simulink model "dx_hand_model"  (R2017b)
settings: Solver=ode3  StartTime=0.0  StopTime=inf  FixedStep=0.01  RelTol=1e-3  EnableMultiTasking=on
InitFcn:
  | cutFreq = 0.1; % T
  | sampleTime = 0.01;
  | filt = tf(1,[cutFreq 1]);
  | filt = c2d(filt,sampleTime);
  | 
  | cutFreq2 = 1;
  | filt2 = tf(1,[cutFreq2 1]);
  | filt2 = c2d(filt2,sampleTime);
  | 
  | cutFreq3 = 0.3;
  | filt3 = tf(1,[cutFreq3 1]);
  | filt3 = c2d(filt3,sampleTime);
  | 
  | update_param = 2;
  | 
  | ampliFactor = 1.60;
  | ampliFactorMiddle = 2.00;
  | ampliFactorDistal = 1;
  | 
  | % Set Hand Address
  | % RightHandAddress = '10.100.39.144';
  | RightHandAddress = '10.24.4.91';
  | Verosim = '10.100.39.22'
  | LeftHandAddress = '10.100.39.22'
  | 
  | max_force = 24; % Newton
model workspace (MAT data in the model file):
  SL_ROS_VariableLengthArrays_MaxSizes : struct (value not decoded)
libraries: robotlib x136, simulink_extras x27, simulink x16, etargetslib x2, dspnetwork x2
(part 16 of 19)

== matlab function dx_hand_model/Thumb/Proximal and Distal Phalanx/Find K ==
  data: PIP input; x_sol output; G2 input; G1 input; s2 input; y_sol output; z_sol output
function [x_sol,y_sol,z_sol] = sysEqn(PIP, G2, G1,s2)
CMC = PIP;
F = G2;
F_1 = G1;
s1 = s2;
CMC1 = CMC(1);
CMC2 = CMC(2);
CMC3 = CMC(3);
F1 = F(1);
F2 =F(2);
F3 = F(3);
F_11 = F_1(1);
F_12 = F_1(2);
F_13 = F_1(3);
%SYSEQNOPTIMIZED
%    [X_SOL,Y_SOL,Z_SOL] = SYSEQNOPTIMIZED(CMC1,CMC2,CMC3,F1,F2,F3,F_11,F_12,F_13,S1)

%    This function was generated by the Symbolic Math Toolbox version 8.0.
%    24-Jan-2018 17:02:07

t2 = CMC1.^2;
t3 = CMC2.^2;
t4 = F1.^2;
t5 = F2.^2;
t6 = F3.^2;
t7 = CMC3.^2;
t8 = s1.^2;
t21 = CMC1.*F1.*2.0;
t22 = CMC2.*F2.*2.0;
t23 = CMC3.*F3.*2.0;
t9 = t2+t3+t4+t5+t6+t7-t21-t22-t23;
t25 = F3.*t2;
t26 = F3.*t3;
t27 = CMC3.*t6.*2.0;
t28 = F3.*t7;
t29 = F3.*t4;
t30 = F3.*t5;
t31 = CMC3.*t8;
t32 = F3.*t8;
t33 = CMC1.*F1.*F3.*2.0;
t34 = CMC2.*F2.*F3.*2.0;
t1256 = F3.*t6;
t10 = t25+t26-t27+t28+t29+t30+t31-t32-t33-t34+t1256;
t11 = t2.^2;
t12 = t4.^2;
t13 = t6.^2;
t14 = t5.^2;
t15 = t3.^2;
t16 = t7.^2;
t17 = F_11.^2;
t18 = F_13.^2;
t19 = F_12.^2;
t20 = t8.^2;
t24 = 1.0./t9.^2;
t35 = t10.^2;
t36 = t24.*t35;
t37 = t2.*t14;
t38 = t3.*t12;
t39 = t5.*t11;
t40 = t4.*t15;
t41 = t2.*t13;
t42 = t6.*t11;
t43 = t7.*t12;
t44 = t4.*t16;
t45 = t3.*t13;
t46 = t7.*t14;
t47 = t6.*t15;
t48 = t5.*t16;
t49 = t11.*t19;
t50 = t15.*t17;
t51 = t11.*t18;
t52 = t16.*t17;
t53 = t15.*t18;
t54 = t16.*t19;
t55 = t12.*t19;
t56 = t14.*t17;
t57 = t12.*t18;
t58 = t13.*t17;
t59 = t14.*t18;
t60 = t13.*t19;
t61 = t2.*t3.*t4;
t62 = t2.*t3.*t5;
t63 = t2.*t4.*t7;
t64 = t2.*t3.*t6.*2.0;
t65 = t2.*t5.*t7.*2.0;
t66 = t3.*t4.*t7.*2.0;
t67 = t2.*t6.*t7;
t68 = t3.*t5.*t7;
t69 = t3.*t6.*t7;
t70 = t2.*t3.*t17;
t71 = t2.*t3.*t19;
t72 = t2.*t7.*t17;
t73 = t2.*t3.*t18.*2.0;
t74 = t2.*t7.*t19.*2.0;
t75 = t3.*t7.*t17.*2.0;
t76 = t2.*t7.*t18;
t77 = t3.*t7.*t19;
t78 = t3.*t7.*t18;
t79 = t2.*t4.*t5;
t80 = t2.*t4.*t6;
t81 = t3.*t4.*t5;
t82 = t2.*t5.*t6.*2.0;
t83 = t3.*t4.*t6.*2.0;
t84 = t4.*t5.*t7.*2.0;
t85 = t3.*t5.*t6;
t86 = t4.*t6.*t7;
t87 = t5.*t6.*t7;
t88 = t2.*t4.*t19.*6.0;
t89 = t2.*t5.*t17;
t90 = t3.*t4.*t17;
t91 = t2.*t4.*t18.*6.0;
t92 = t2.*t5.*t19;
t93 = t2.*t6.*t17;
t94 = t3.*t4.*t19;
t95 = t3.*t5.*t17.*6.0;
t96 = t4.*t7.*t17;
t97 = t2.*t5.*t18.*2.0;
t98 = t2.*t6.*t19.*2.0;
t99 = t3.*t4.*t18.*2.0;
t100 = t3.*t6.*t17.*2.0;
t101 = t4.*t7.*t19.*2.0;
t102 = t5.*t7.*t17.*2.0;
t103 = t2.*t6.*t18;
t104 = t3.*t5.*t18.*6.0;
t105 = t3.*t6.*t19;
t106 = t4.*t7.*t18;
t107 = t5.*t7.*t19;
t108 = t6.*t7.*t17.*6.0;
t109 = t3.*t6.*t18;
t110 = t5.*t7.*t18;
t111 = t6.*t7.*t19.*6.0;
t112 = t4.*t5.*t17;
t113 = t4.*t5.*t19;
t114 = t4.*t6.*t17;
t115 = t4.*t5.*t18.*2.0;
t116 = t4.*t6.*t19.*2.0;
t117 = t5.*t6.*t17.*2.0;
t118 = t4.*t6.*t18;
t119 = t5.*t6.*t19;
t120 = t5.*t6.*t18;
t121 = CMC1.*F1.*t3.*t5.*4.0;
t122 = CMC2.*F2.*t2.*t4.*4.0;
t123 = CMC1.*F1.*t6.*t7.*4.0;
t124 = CMC3.*F3.*t2.*t4.*4.0;
t125 = CMC2.*F2.*t6.*t7.*4.0;
t126 = CMC3.*F3.*t3.*t5.*4.0;
t127 = CMC1.*F_11.*t3.*t4.*4.0;
t128 = CMC1.*F_11.*t4.*t7.*4.0;
t129 = CMC2.*F_12.*t2.*t5.*4.0;
t130 = CMC2.*F_12.*t5.*t7.*4.0;
t131 = CMC3.*F_13.*t2.*t6.*4.0;
t132 = CMC3.*F_13.*t3.*t6.*4.0;
t133 = F1.*F_11.*t2.*t5.*4.0;
t134 = F1.*F_11.*t2.*t6.*4.0;
t135 = F2.*F_12.*t3.*t4.*4.0;
t136 = F2.*F_12.*t3.*t6.*4.0;
t137 = F3.*F_13.*t4.*t7.*4.0;
t138 = F3.*F_13.*t5.*t7.*4.0;
t139 = CMC1.*CMC2.*F1.*F_12.*t4.*6.0;
t140 = CMC1.*CMC2.*F2.*F_11.*t5.*6.0;
t141 = CMC1.*CMC2.*F1.*F_12.*t3.*2.0;
t142 = CMC1.*CMC2.*F2.*F_11.*t3.*2.0;
t143 = CMC1.*CMC2.*F1.*F_12.*t2.*2.0;
t144 = CMC1.*CMC2.*F2.*F_11.*t2.*2.0;
t145 = CMC1.*CMC3.*F1.*F_13.*t4.*6.0;
t146 = CMC1.*CMC3.*F3.*F_11.*t6.*6.0;
t147 = CMC1.*CMC3.*F1.*F_13.*t7.*2.0;
t148 = CMC1.*CMC3.*F3.*F_11.*t7.*2.0;
t149 = CMC1.*CMC3.*F1.*F_13.*t2.*2.0;
t150 = CMC1.*CMC3.*F3.*F_11.*t2.*2.0;
t151 = CMC2.*CMC3.*F2.*F_13.*t5.*6.0;
t152 = CMC2.*CMC3.*F3.*F_12.*t6.*6.0;
t153 = CMC2.*CMC3.*F2.*F_13.*t7.*2.0;
t154 = CMC2.*CMC3.*F3.*F_12.*t7.*2.0;
t155 = CMC2.*CMC3.*F2.*F_13.*t3.*2.0;
t156 = CMC2.*CMC3.*F3.*F_12.*t3.*2.0;
t157 = CMC1.*F1.*F2.*F_12.*t5.*2.0;
t158 = CMC1.*F1.*F2.*F_12.*t4.*2.0;
t159 = CMC2.*F1.*F2.*F_11.*t5.*2.0;
t160 = CMC2.*F1.*F2.*F_11.*t4.*2.0;
t161 = CMC1.*F1.*F2.*F_12.*t2.*6.0;
t162 = CMC2.*F1.*F2.*F_11.*t3.*6.0;
t163 = CMC1.*F1.*F3.*F_13.*t6.*2.0;
t164 = CMC1.*F1.*F3.*F_13.*t4.*2.0;
t165 = CMC3.*F1.*F3.*F_11.*t6.*2.0;
t166 = CMC3.*F1.*F3.*F_11.*t4.*2.0;
t167 = CMC1.*F1.*F3.*F_13.*t2.*6.0;
t168 = CMC3.*F1.*F3.*F_11.*t7.*6.0;
t169 = CMC2.*F2.*F3.*F_13.*t6.*2.0;
t170 = CMC2.*F2.*F3.*F_13.*t5.*2.0;
t171 = CMC3.*F2.*F3.*F_12.*t6.*2.0;
t172 = CMC3.*F2.*F3.*F_12.*t5.*2.0;
t173 = CMC2.*F2.*F3.*F_13.*t3.*6.0;
t174 = CMC3.*F2.*F3.*F_12.*t7.*6.0;
t175 = CMC1.*F2.*F_11.*F_12.*t5.*2.0;
t176 = CMC2.*F1.*F_11.*F_12.*t4.*2.0;
t177 = CMC1.*F2.*F_11.*F_12.*t2.*2.0;
t178 = CMC2.*F1.*F_11.*F_12.*t3.*2.0;
t179 = CMC1.*F3.*F_11.*F_13.*t6.*2.0;
t180 = CMC3.*F1.*F_11.*F_13.*t4.*2.0;
t181 = CMC1.*F3.*F_11.*F_13.*t2.*2.0;
t182 = CMC3.*F1.*F_11.*F_13.*t7.*2.0;
t183 = CMC2.*F3.*F_12.*F_13.*t6.*2.0;
t184 = CMC3.*F2.*F_12.*F_13.*t5.*2.0;
t185 = CMC2.*F3.*F_12.*F_13.*t3.*2.0;
t186 = CMC3.*F2.*F_12.*F_13.*t7.*2.0;
t187 = CMC1.*CMC2.*F1.*F_12.*t7.*2.0;
t188 = CMC1.*CMC2.*F2.*F_11.*t7.*2.0;
t189 = CMC1.*CMC3.*F1.*F_13.*t3.*2.0;
t190 = CMC1.*CMC3.*F3.*F_11.*t3.*2.0;
t191 = CMC2.*CMC3.*F2.*F_13.*t2.*2.0;
t192 = CMC2.*CMC3.*F3.*F_12.*t2.*2.0;
t193 = CMC1.*CMC2.*F1.*F2.*t17.*4.0;
t194 = CMC1.*CMC2.*F1.*F2.*t19.*4.0;
t195 = CMC1.*CMC2.*F1.*F2.*t18.*8.0;
t196 = CMC1.*CMC2.*F1.*F_12.*t6.*6.0;
t197 = CMC1.*CMC2.*F2.*F_11.*t6.*6.0;
t198 = CMC1.*CMC3.*F1.*F3.*t17.*4.0;
t199 = CMC1.*F1.*F2.*F_12.*t7.*6.0;
t200 = CMC2.*F1.*F2.*F_11.*t7.*6.0;
t201 = CMC1.*CMC3.*F1.*F3.*t19.*8.0;
t202 = CMC1.*CMC3.*F1.*F_13.*t5.*6.0;
t203 = CMC1.*CMC3.*F3.*F_11.*t5.*6.0;
t204 = CMC1.*F1.*F3.*F_13.*t3.*6.0;
t205 = CMC3.*F1.*F3.*F_11.*t3.*6.0;
t206 = CMC1.*CMC3.*F1.*F3.*t18.*4.0;
t207 = CMC2.*CMC3.*F2.*F3.*t17.*8.0;
t208 = CMC2.*CMC3.*F2.*F_13.*t4.*6.0;
t209 = CMC2.*CMC3.*F3.*F_12.*t4.*6.0;
t210 = CMC2.*F2.*F3.*F_13.*t2.*6.0;
t211 = CMC3.*F2.*F3.*F_12.*t2.*6.0;
t212 = CMC2.*CMC3.*F2.*F3.*t19.*4.0;
t213 = CMC2.*CMC3.*F2.*F3.*t18.*4.0;
t214 = CMC2.*F1.*F_11.*F_12.*t2.*6.0;
t215 = CMC1.*F2.*F_11.*F_12.*t3.*6.0;
t216 = CMC1.*F2.*F_11.*F_12.*t7.*2.0;
t217 = CMC2.*F1.*F_11.*F_12.*t7.*2.0;
t218 = CMC3.*F1.*F_11.*F_13.*t2.*6.0;
t219 = CMC1.*F3.*F_11.*F_13.*t3.*2.0;
t220 = CMC3.*F1.*F_11.*F_13.*t3.*2.0;
t221 = CMC1.*F3.*F_11.*F_13.*t7.*6.0;
t222 = CMC2.*F3.*F_12.*F_13.*t2.*2.0;
t223 = CMC3.*F2.*F_12.*F_13.*t2.*2.0;
t224 = CMC3.*F2.*F_12.*F_13.*t3.*6.0;
t225 = CMC2.*F3.*F_12.*F_13.*t7.*6.0;
t226 = CMC1.*F1.*F2.*F_12.*t6.*2.0;
t227 = CMC2.*F1.*F2.*F_11.*t6.*2.0;
t228 = CMC1.*F1.*F3.*F_13.*t5.*2.0;
t229 = CMC3.*F1.*F3.*F_11.*t5.*2.0;
t230 = CMC2.*F2.*F3.*F_13.*t4.*2.0;
t231 = CMC3.*F2.*F3.*F_12.*t4.*2.0;
t232 = CMC1.*F2.*F_11.*F_12.*t4.*6.0;
t233 = CMC2.*F1.*F_11.*F_12.*t5.*6.0;
t234 = CMC1.*F2.*F_11.*F_12.*t6.*2.0;
t235 = CMC1.*F3.*F_11.*F_13.*t4.*6.0;
t236 = CMC2.*F1.*F_11.*F_12.*t6.*2.0;
t237 = CMC1.*F3.*F_11.*F_13.*t5.*2.0;
t238 = CMC3.*F1.*F_11.*F_13.*t5.*2.0;
t239 = CMC2.*F3.*F_12.*F_13.*t4.*2.0;
t240 = CMC3.*F1.*F_11.*F_13.*t6.*6.0;
t241 = CMC3.*F2.*F_12.*F_13.*t4.*2.0;
t242 = CMC2.*F3.*F_12.*F_13.*t5.*6.0;
t243 = CMC3.*F2.*F_12.*F_13.*t6.*6.0;
t244 = CMC1.*F1.*F2.*F3.*F_12.*F_13.*4.0;
t245 = CMC2.*F1.*F2.*F3.*F_11.*F_13.*4.0;
t246 = CMC3.*F1.*F2.*F3.*F_11.*F_12.*4.0;
t247 = CMC1.*CMC2.*CMC3.*F1.*F2.*F3.*1.2e1;
t248 = CMC1.*CMC2.*CMC3.*F1.*F_12.*F_13.*4.0;
t249 = CMC1.*CMC2.*CMC3.*F2.*F_11.*F_13.*4.0;
t250 = CMC1.*CMC2.*CMC3.*F3.*F_11.*F_12.*4.0;
t633 = CMC1.*F_11.*t14.*2.0;
t634 = F1.*F_11.*t15.*2.0;
t635 = CMC1.*F_11.*t13.*2.0;
t636 = CMC2.*F_12.*t12.*2.0;
t637 = F2.*F_12.*t11.*2.0;
t638 = F1.*F_11.*t16.*2.0;
t639 = CMC2.*F_12.*t13.*2.0;
t640 = CMC3.*F_13.*t12.*2.0;
t641 = F3.*F_13.*t11.*2.0;
t642 = F2.*F_12.*t16.*2.0;
t643 = CMC3.*F_13.*t14.*2.0;
t644 = F3.*F_13.*t15.*2.0;
t645 = CMC1.*F1.*t3.*t4.*2.0;
t646 = CMC1.*F1.*t4.*t7.*2.0;
t647 = CMC2.*F2.*t2.*t5.*2.0;
t648 = CMC2.*F2.*t5.*t7.*2.0;
t649 = CMC3.*F3.*t2.*t6.*2.0;
t650 = CMC3.*F3.*t3.*t6.*2.0;
t651 = CMC1.*F1.*t2.*t5.*2.0;
t652 = CMC1.*F1.*t2.*t6.*2.0;
t653 = CMC2.*F2.*t3.*t4.*2.0;
t654 = CMC2.*F2.*t3.*t6.*2.0;
t655 = CMC3.*F3.*t4.*t7.*2.0;
t656 = CMC3.*F3.*t5.*t7.*2.0;
t657 = CMC1.*F1.*t4.*t19.*4.0;
t658 = CMC1.*F1.*t2.*t19.*4.0;
t659 = CMC1.*F_11.*t2.*t5.*2.0;
t660 = F1.*F_11.*t3.*t4.*2.0;
t661 = CMC1.*F1.*t4.*t18.*4.0;
t662 = CMC2.*F2.*t5.*t17.*4.0;
t663 = F2.*F_12.*t2.*t5.*2.0;
t664 = CMC1.*F1.*t2.*t18.*4.0;
t665 = CMC1.*F_11.*t2.*t6.*2.0;
t666 = CMC2.*F2.*t3.*t17.*4.0;
t667 = CMC2.*F_12.*t3.*t4.*2.0;
t668 = F1.*F_11.*t4.*t7.*2.0;
t669 = CMC2.*F2.*t5.*t18.*4.0;
t670 = CMC3.*F3.*t6.*t17.*4.0;
t671 = F3.*F_13.*t2.*t6.*2.0;
t672 = CMC2.*F2.*t3.*t18.*4.0;
t673 = CMC2.*F_12.*t3.*t6.*2.0;
t674 = F2.*F_12.*t5.*t7.*2.0;
t675 = CMC3.*F3.*t7.*t17.*4.0;
t676 = CMC3.*F_13.*t4.*t7.*2.0;
t677 = CMC3.*F3.*t6.*t19.*4.0;
t678 = F3.*F_13.*t3.*t6.*2.0;
t679 = CMC3.*F3.*t7.*t19.*4.0;
t680 = CMC3.*F_13.*t5.*t7.*2.0;
t681 = CMC1.*F1.*t3.*t6.*2.0;
t682 = CMC1.*F1.*t5.*t7.*2.0;
t683 = CMC2.*F2.*t4.*t7.*2.0;
t684 = CMC2.*F2.*t2.*t6.*2.0;
t685 = CMC3.*F3.*t2.*t5.*2.0;
t686 = CMC3.*F3.*t3.*t4.*2.0;
t687 = CMC1.*F1.*t3.*t17.*2.0;
t688 = F1.*F_11.*t2.*t3.*2.0;
t689 = CMC1.*F1.*t3.*t19.*2.0;
t690 = CMC1.*F_11.*t3.*t5.*6.0;
t691 = CMC1.*F1.*t7.*t17.*2.0;
t692 = CMC2.*F2.*t2.*t17.*2.0;
t693 = CMC2.*F_12.*t2.*t4.*6.0;
t694 = F1.*F_11.*t2.*t7.*2.0;
t695 = CMC1.*F1.*t3.*t18.*4.0;
t696 = CMC1.*F_11.*t3.*t6.*2.0;
t697 = CMC1.*F1.*t7.*t19.*4.0;
t698 = CMC1.*F_11.*t5.*t7.*2.0;
t699 = CMC2.*F2.*t2.*t19.*2.0;
t700 = F2.*F_12.*t2.*t3.*2.0;
t701 = F1.*F_11.*t3.*t7.*4.0;
t702 = CMC1.*F1.*t7.*t18.*2.0;
t703 = CMC1.*F_11.*t6.*t7.*6.0;
t704 = CMC2.*F2.*t7.*t17.*4.0;
t705 = CMC2.*F_12.*t4.*t7.*2.0;
t706 = CMC2.*F2.*t2.*t18.*4.0;
t707 = CMC2.*F_12.*t2.*t6.*2.0;
t708 = CMC3.*F3.*t2.*t17.*2.0;
t709 = CMC3.*F_13.*t2.*t4.*6.0;
t710 = F2.*F_12.*t2.*t7.*4.0;
t711 = CMC2.*F2.*t7.*t19.*2.0;
t712 = CMC3.*F3.*t2.*t19.*4.0;
t713 = CMC3.*F_13.*t2.*t5.*2.0;
t714 = F3.*F_13.*t2.*t3.*4.0;
t715 = CMC3.*F3.*t3.*t17.*4.0;
t716 = CMC3.*F_13.*t3.*t4.*2.0;
t717 = F2.*F_12.*t3.*t7.*2.0;
t718 = CMC2.*F2.*t7.*t18.*2.0;
t719 = CMC2.*F_12.*t6.*t7.*6.0;
t720 = CMC3.*F3.*t2.*t18.*2.0;
t721 = F3.*F_13.*t2.*t7.*2.0;
t722 = CMC3.*F3.*t3.*t19.*2.0;
t723 = CMC3.*F_13.*t3.*t5.*6.0;
t724 = CMC3.*F3.*t3.*t18.*2.0;
t725 = F3.*F_13.*t3.*t7.*2.0;
t726 = CMC1.*F1.*t5.*t17.*2.0;
t727 = CMC1.*F_11.*t4.*t5.*2.0;
t728 = CMC1.*F1.*t5.*t19.*2.0;
t729 = CMC1.*F1.*t6.*t17.*2.0;
t730 = CMC1.*F_11.*t4.*t6.*2.0;
t731 = CMC2.*F2.*t4.*t17.*2.0;
t732 = F2.*F_12.*t2.*t4.*6.0;
t733 = F1.*F_11.*t3.*t5.*6.0;
t734 = CMC1.*F1.*t5.*t18.*4.0;
t735 = CMC1.*F1.*t6.*t19.*4.0;
t736 = CMC1.*F_11.*t5.*t6.*4.0;
t737 = CMC2.*F2.*t4.*t19.*2.0;
t738 = CMC2.*F_12.*t4.*t5.*2.0;
t739 = F1.*F_11.*t3.*t6.*2.0;
t740 = F1.*F_11.*t5.*t7.*2.0;
t741 = CMC1.*F1.*t6.*t18.*2.0;
t742 = CMC2.*F2.*t6.*t17.*4.0;
t743 = CMC2.*F2.*t4.*t18.*4.0;
t744 = CMC2.*F_12.*t4.*t6.*4.0;
t745 = CMC3.*F3.*t4.*t17.*2.0;
t746 = F2.*F_12.*t2.*t6.*2.0;
t747 = F3.*F_13.*t2.*t4.*6.0;
t748 = F1.*F_11.*t6.*t7.*6.0;
t749 = F2.*F_12.*t4.*t7.*2.0;
t750 = CMC2.*F2.*t6.*t19.*2.0;
t751 = CMC2.*F_12.*t5.*t6.*2.0;
t752 = CMC3.*F3.*t4.*t19.*4.0;
t753 = CMC3.*F_13.*t4.*t5.*4.0;
t754 = CMC3.*F3.*t5.*t17.*4.0;
t755 = F3.*F_13.*t2.*t5.*2.0;
t756 = F3.*F_13.*t3.*t4.*2.0;
t757 = CMC2.*F2.*t6.*t18.*2.0;
t758 = CMC3.*F3.*t4.*t18.*2.0;
t759 = CMC3.*F_13.*t4.*t6.*2.0;
t760 = CMC3.*F3.*t5.*t19.*2.0;
t761 = F3.*F_13.*t3.*t5.*6.0;
t762 = F2.*F_12.*t6.*t7.*6.0;
t763 = CMC3.*F3.*t5.*t18.*2.0;
t764 = CMC3.*F_13.*t5.*t6.*2.0;
t765 = CMC1.*CMC2.*F1.*F2.*t5.*2.0;
t766 = CMC1.*CMC2.*F1.*F2.*t4.*2.0;
t767 = CMC1.*CMC2.*F1.*F2.*t3.*2.0;
t768 = CMC1.*CMC2.*F1.*F2.*t2.*2.0;
t769 = CMC1.*CMC3.*F1.*F3.*t6.*2.0;
t770 = CMC1.*CMC3.*F1.*F3.*t4.*2.0;
t771 = CMC1.*CMC3.*F1.*F3.*t7.*2.0;
t772 = CMC1.*CMC3.*F1.*F3.*t2.*2.0;
t773 = CMC2.*CMC3.*F2.*F3.*t6.*2.0;
t774 = CMC2.*CMC3.*F2.*F3.*t5.*2.0;
t775 = CMC2.*CMC3.*F2.*F3.*t7.*2.0;
t776 = CMC2.*CMC3.*F2.*F3.*t3.*2.0;
t777 = CMC1.*CMC2.*F_11.*F_12.*t3.*2.0;
t778 = CMC1.*CMC2.*F_11.*F_12.*t2.*2.0;
t779 = CMC1.*CMC3.*F_11.*F_13.*t7.*2.0;
t780 = CMC1.*CMC3.*F_11.*F_13.*t2.*2.0;
t781 = CMC2.*CMC3.*F_12.*F_13.*t7.*2.0;
t782 = CMC2.*CMC3.*F_12.*F_13.*t3.*2.0;
t783 = F1.*F2.*F_11.*F_12.*t5.*2.0;
t784 = F1.*F2.*F_11.*F_12.*t4.*2.0;
t785 = F1.*F3.*F_11.*F_13.*t6.*2.0;
t786 = F1.*F3.*F_11.*F_13.*t4.*2.0;
t787 = F2.*F3.*F_12.*F_13.*t6.*2.0;
t788 = F2.*F3.*F_12.*F_13.*t5.*2.0;
t789 = CMC1.*CMC2.*F1.*F2.*t7.*2.0;
t790 = CMC1.*CMC3.*F1.*F3.*t3.*2.0;
t791 = CMC2.*CMC3.*F2.*F3.*t2.*2.0;
t792 = CMC1.*CMC2.*F_11.*F_12.*t7.*2.0;
t793 = CMC1.*CMC3.*F_11.*F_13.*t3.*2.0;
t794 = CMC2.*CMC3.*F_12.*F_13.*t2.*2.0;
t795 = CMC1.*CMC2.*F1.*F2.*t6.*2.0;
t796 = CMC1.*CMC3.*F1.*F3.*t5.*2.0;
t797 = CMC2.*CMC3.*F2.*F3.*t4.*2.0;
t798 = CMC1.*CMC2.*F2.*F_11.*t4.*2.0;
t799 = CMC2.*F1.*F2.*F_11.*t2.*2.0;
t800 = CMC1.*CMC2.*F1.*F_12.*t5.*2.0;
t801 = CMC1.*F1.*F2.*F_12.*t3.*2.0;
t802 = CMC1.*CMC3.*F3.*F_11.*t4.*2.0;
t803 = CMC3.*F1.*F3.*F_11.*t2.*2.0;
t804 = CMC1.*CMC3.*F1.*F_13.*t6.*2.0;
t805 = CMC1.*F1.*F3.*F_13.*t7.*2.0;
t806 = CMC2.*CMC3.*F3.*F_12.*t5.*2.0;
t807 = CMC3.*F2.*F3.*F_12.*t3.*2.0;
t808 = CMC2.*CMC3.*F2.*F_13.*t6.*2.0;
t809 = CMC2.*F2.*F3.*F_13.*t7.*2.0;
t810 = CMC1.*CMC2.*F_11.*F_12.*t4.*6.0;
t811 = CMC1.*CMC2.*F_11.*F_12.*t5.*6.0;
t812 = CMC1.*CMC2.*F_11.*F_12.*t6.*2.0;
t813 = CMC1.*CMC3.*F_11.*F_13.*t4.*6.0;
t814 = CMC1.*CMC3.*F_11.*F_13.*t5.*2.0;
t815 = CMC1.*CMC3.*F_11.*F_13.*t6.*6.0;
t816 = CMC2.*CMC3.*F_12.*F_13.*t4.*2.0;
t817 = CMC2.*CMC3.*F_12.*F_13.*t5.*6.0;
t818 = CMC2.*CMC3.*F_12.*F_13.*t6.*6.0;
t819 = F1.*F2.*F_11.*F_12.*t2.*6.0;
t820 = F1.*F2.*F_11.*F_12.*t3.*6.0;
t821 = F1.*F3.*F_11.*F_13.*t2.*6.0;
t822 = F1.*F2.*F_11.*F_12.*t7.*2.0;
t823 = F1.*F3.*F_11.*F_13.*t3.*2.0;
t824 = F2.*F3.*F_12.*F_13.*t2.*2.0;
t825 = F1.*F3.*F_11.*F_13.*t7.*6.0;
t826 = F2.*F3.*F_12.*F_13.*t3.*6.0;
t827 = F2.*F3.*F_12.*F_13.*t7.*6.0;
t828 = F1.*F2.*F_11.*F_12.*t6.*2.0;
t829 = F1.*F3.*F_11.*F_13.*t5.*2.0;
t830 = F2.*F3.*F_12.*F_13.*t4.*2.0;
t831 = CMC1.*CMC2.*CMC3.*F1.*F2.*F_13.*8.0;
t832 = CMC1.*CMC2.*CMC3.*F1.*F3.*F_12.*8.0;
t833 = CMC1.*CMC2.*CMC3.*F2.*F3.*F_11.*8.0;
t834 = CMC1.*CMC2.*F1.*F2.*F3.*F_13.*8.0;
t835 = CMC1.*CMC3.*F1.*F2.*F3.*F_12.*8.0;
t836 = CMC2.*CMC3.*F1.*F2.*F3.*F_11.*8.0;
t837 = CMC1.*CMC2.*F1.*F3.*F_12.*F_13.*4.0;
t838 = CMC1.*CMC2.*F2.*F3.*F_11.*F_13.*4.0;
t839 = CMC1.*CMC3.*F1.*F2.*F_12.*F_13.*4.0;
t840 = CMC1.*CMC3.*F2.*F3.*F_11.*F_12.*4.0;
t841 = CMC2.*CMC3.*F1.*F2.*F_11.*F_13.*4.0;
t842 = CMC2.*CMC3.*F1.*F3.*F_11.*F_12.*4.0;
t251 = t37+t38+t39+t40+t41+t42+t43+t44+t45+t46+t47+t48+t49+t50+t51+t52+t53+t54+t55+t56+t57+t58+t59+t60+t61+t62+t63+t64+t65+t66+t67+t68+t69+t70+t71+t72+t73+t74+t75+t76+t77+t78+t79+t80+t81+t82+t83+t84+t85+t86+t87+t88+t89+t90+t91+t92+t93+t94+t95+t96+t97+t98+t99+t100+t101+t102+t103+t104+t105+t106+t107+t108+t109+t110+t111+t112+t113+t114+t115+t116+t117+t118+t119+t120+t121+t122+t123+t124+t125+t126+t127+t128+t129+t130+t131+t132+t133+t134+t135+t136+t137+t138+t139+t140+t141+t142+t143+t144+t145+t146+t147+t148+t149+t150+t151+t152+t153+t154+t155+t156+t157+t158+t159+t160+t161+t162+t163+t164+t165+t166+t167+t168+t169+t170+t171+t172+t173+t174+t175+t176+t177+t178+t179+t180+t181+t182+t183+t184+t185+t186+t187+t188+t189+t190+t191+t192+t193+t194+t195+t196+t197+t198+t199+t200+t201+t202+t203+t204+t205+t206+t207+t208+t209+t210+t211+t212+t213+t214+t215+t216+t217+t218+t219+t220+t221+t222+t223+t224+t225+t226+t227+t228+t229+t230+t231+t232+t233+t234+t235+t236+t237+t238+t239+t240+t241+t242+t243+t244+t245+t246+t247+t248+t249+t250-t633-t634-t635-t636-t637-t638-t639-t640-t641-t642-t643-t644-t645-t646-t647-t648-t649-t650-t651-t652-t653-t654-t655-t656-t657-t658-t659-t660-t661-t662-t663-t664-t665-t666-t667-t668-t669-t670-t671-t672-t673-t674-t675-t676-t677-t678-t679-t680-t681-t682-t683-t684-t685-t686-t687-t688-t689-t690-t691-t692-t693-t694-t695-t696-t697-t698-t699-t700-t701-t702-t703-t704-t705-t706-t707-t708-t709-t710-t711-t712-t713-t714-t715-t716-t717-t718-t719-t720-t721-t722-t723-t724-t725-t726-t727-t728-t729-t730-t731-t732-t733-t734-t735-t736-t737-t738-t739-t740-t741-t742-t743-t744-t745-t746-t747-t748-t749-t750-t751-t752-t753-t754-t755-t756-t757-t758-t759-t760-t761-t762-t763-t764-t765-t766-t767-t768-t769-t770-t771-t772-t773-t774-t775-t776-t777-t778-t779-t780-t781-t782-t783-t784-t785-t786-t787-t788-t789-t790-t791-t792-t793-t794-t795-t796-t797-t798-t799-t800-t801-t802-t803-t804-t805-t806-t807-t808-t809-t810-t811-t812-t813-t814-t815-t816-t817-t818-t819-t820-t821-t822-t823-t824-t825-t826-t827-t828-t829-t830-t831-t832-t833-t834-t835-t836-t837-t838-t839-t840-t841-t842;
t252 = 1.0./t251;
t253 = t2.*t6.*t13;
t254 = t11.*t13;
t255 = t3.*t6.*t13;
t256 = t13.*t15;
t257 = t6.*t13.*t17;
t258 = t6.*t13.*t19;
t259 = t2.*t3.*t13.*2.0;
t260 = t2.*t7.*t13;
t261 = t3.*t7.*t13;
t262 = t2.*t4.*t13;
t263 = t2.*t5.*t13.*2.0;
t264 = t2.*t6.*t14;
t265 = t3.*t4.*t13.*2.0;
t266 = t3.*t6.*t12;
t267 = t5.*t6.*t11;
t268 = t4.*t6.*t15;
t269 = t3.*t5.*t13;
t270 = t4.*t7.*t13;
t271 = t6.*t7.*t12;
t272 = t4.*t6.*t16;
t273 = t5.*t7.*t13;
t274 = t6.*t7.*t14;
t275 = t5.*t6.*t16;
t276 = t2.*t13.*t17;
t277 = t2.*t13.*t19.*2.0;
t278 = t3.*t13.*t17.*2.0;
t279 = t6.*t11.*t19;
t280 = t6.*t15.*t17;
t281 = t2.*t13.*t18;
t282 = t3.*t13.*t19;
t283 = t6.*t11.*t18;
t284 = t7.*t13.*t17.*6.0;
t285 = t6.*t16.*t17;
t286 = t3.*t13.*t18;
t287 = t7.*t13.*t19.*6.0;
t288 = t6.*t15.*t18;
t289 = t6.*t16.*t19;
t290 = t4.*t13.*t17;
t291 = t4.*t13.*t19.*2.0;
t292 = t5.*t13.*t17.*2.0;
t293 = t6.*t12.*t19;
t294 = t6.*t14.*t17;
t295 = t4.*t13.*t18;
t296 = t5.*t13.*t19;
t297 = t6.*t12.*t18;
t298 = t5.*t13.*t18;
t299 = t6.*t14.*t18;
t300 = t2.*t6.*t20;
t301 = t4.*t7.*t20;
t302 = t3.*t6.*t20;
t303 = t5.*t7.*t20;
t304 = t2.*t18.*t20;
t305 = t7.*t17.*t20;
t306 = t3.*t18.*t20;
t307 = t7.*t19.*t20;
t308 = t4.*t18.*t20;
t309 = t6.*t17.*t20;
t310 = t5.*t18.*t20;
t311 = t6.*t19.*t20;
t312 = CMC1.*F1.*t7.*t13.*4.0;
t313 = CMC2.*F2.*t7.*t13.*4.0;
t314 = CMC1.*CMC3.*F3.*F_11.*t6.*t7.*2.0;
t315 = CMC1.*CMC3.*F3.*F_11.*t2.*t6.*2.0;
t316 = CMC2.*CMC3.*F3.*F_12.*t6.*t7.*2.0;
t317 = CMC3.*F_13.*t2.*t13.*4.0;
t318 = CMC2.*CMC3.*F3.*F_12.*t3.*t6.*2.0;
t319 = CMC3.*F_13.*t3.*t13.*4.0;
t320 = F1.*F_11.*t2.*t13.*4.0;
t321 = CMC1.*F1.*F3.*F_13.*t4.*t6.*2.0;
t322 = CMC3.*F1.*F3.*F_11.*t4.*t6.*2.0;
t323 = CMC1.*F1.*F3.*F_13.*t2.*t6.*6.0;
t324 = CMC3.*F1.*F3.*F_11.*t6.*t7.*6.0;
t325 = F2.*F_12.*t3.*t13.*4.0;
t326 = CMC2.*F2.*F3.*F_13.*t5.*t6.*2.0;
t327 = CMC3.*F2.*F3.*F_12.*t5.*t6.*2.0;
t328 = CMC2.*F2.*F3.*F_13.*t3.*t6.*6.0;
t329 = CMC3.*F2.*F3.*F_12.*t6.*t7.*6.0;
t330 = CMC1.*F3.*F_11.*F_13.*t2.*t6.*2.0;
t331 = CMC2.*F3.*F_12.*F_13.*t3.*t6.*2.0;
t332 = CMC1.*F_11.*t8.*t13.*4.0;
t333 = CMC2.*F_12.*t8.*t13.*4.0;
t334 = CMC3.*F_13.*t8.*t12.*2.0;
t335 = F3.*F_13.*t8.*t11.*2.0;
t336 = CMC3.*F_13.*t8.*t14.*2.0;
t337 = F3.*F_13.*t8.*t15.*2.0;
t338 = CMC3.*F3.*t2.*t4.*t6.*4.0;
t339 = CMC3.*F3.*t3.*t5.*t6.*4.0;
t340 = F3.*F_13.*t4.*t6.*t7.*4.0;
t341 = F3.*F_13.*t5.*t6.*t7.*4.0;
t342 = CMC1.*F1.*t4.*t7.*t8.*2.0;
t343 = CMC2.*F2.*t5.*t7.*t8.*2.0;
t344 = CMC3.*F3.*t2.*t6.*t8.*2.0;
t345 = CMC3.*F3.*t3.*t6.*t8.*2.0;
t346 = CMC1.*F1.*t2.*t6.*t8.*2.0;
t347 = CMC2.*F2.*t3.*t6.*t8.*2.0;
t348 = CMC3.*F3.*t4.*t7.*t8.*2.0;
t349 = CMC3.*F3.*t5.*t7.*t8.*2.0;
t350 = CMC1.*F1.*t4.*t8.*t18.*4.0;
t351 = CMC1.*F1.*t2.*t8.*t18.*4.0;
t352 = CMC1.*F_11.*t2.*t6.*t8.*2.0;
t353 = F1.*F_11.*t4.*t7.*t8.*2.0;
t354 = CMC2.*F2.*t5.*t8.*t18.*4.0;
t355 = CMC3.*F3.*t6.*t8.*t17.*6.0;
t356 = F3.*F_13.*t2.*t6.*t8.*4.0;
t357 = CMC2.*F2.*t3.*t8.*t18.*4.0;
t358 = CMC2.*F_12.*t3.*t6.*t8.*2.0;
t359 = F2.*F_12.*t5.*t7.*t8.*2.0;
t360 = CMC3.*F3.*t7.*t8.*t17.*2.0;
t361 = CMC3.*F3.*t6.*t8.*t19.*6.0;
t362 = F3.*F_13.*t3.*t6.*t8.*4.0;
t363 = CMC3.*F3.*t7.*t8.*t19.*2.0;
t364 = CMC1.*CMC3.*F3.*F_11.*t13.*6.0;
t365 = CMC2.*CMC3.*F3.*F_12.*t13.*6.0;
t366 = CMC1.*F1.*F3.*F_13.*t13.*2.0;
t367 = CMC3.*F1.*F3.*F_11.*t13.*2.0;
t368 = CMC2.*F2.*F3.*F_13.*t13.*2.0;
t369 = CMC3.*F2.*F3.*F_12.*t13.*2.0;
t370 = CMC1.*F3.*F_11.*F_13.*t13.*2.0;
t371 = CMC2.*F3.*F_12.*F_13.*t13.*2.0;
t372 = t2.*t3.*t4.*t6;
t373 = t2.*t3.*t5.*t6;
t374 = t2.*t4.*t6.*t7;
t375 = t2.*t5.*t6.*t7.*2.0;
t376 = t3.*t4.*t6.*t7.*2.0;
t377 = t3.*t5.*t6.*t7;
t378 = t2.*t3.*t6.*t17;
t379 = t2.*t3.*t6.*t19;
t380 = t2.*t6.*t7.*t17;
t381 = t2.*t3.*t6.*t18.*2.0;
t382 = t2.*t6.*t7.*t19.*2.0;
t383 = t3.*t6.*t7.*t17.*2.0;
t384 = t2.*t6.*t7.*t18;
t385 = t3.*t6.*t7.*t19;
t386 = t3.*t6.*t7.*t18;
t387 = t2.*t4.*t5.*t6;
t388 = t3.*t4.*t5.*t6;
t389 = t4.*t5.*t6.*t7.*2.0;
t390 = t2.*t4.*t6.*t19.*6.0;
t391 = t2.*t5.*t6.*t17;
t392 = t3.*t4.*t6.*t17;
t393 = t2.*t4.*t6.*t18.*6.0;
t394 = t2.*t5.*t6.*t19;
t395 = t3.*t4.*t6.*t19;
t396 = t3.*t5.*t6.*t17.*6.0;
t397 = t4.*t6.*t7.*t17;
t398 = t2.*t5.*t6.*t18.*2.0;
t399 = t3.*t4.*t6.*t18.*2.0;
t400 = t4.*t6.*t7.*t19.*2.0;
t401 = t5.*t6.*t7.*t17.*2.0;
t402 = t3.*t5.*t6.*t18.*6.0;
t403 = t4.*t6.*t7.*t18;
t404 = t5.*t6.*t7.*t19;
t405 = t5.*t6.*t7.*t18;
t406 = t4.*t5.*t6.*t17;
t407 = t4.*t5.*t6.*t19;
t408 = t4.*t5.*t6.*t18.*2.0;
t409 = CMC1.*F1.*t3.*t6.*t8.*2.0;
t410 = CMC1.*F1.*t5.*t7.*t8.*2.0;
t411 = CMC2.*F2.*t4.*t7.*t8.*2.0;
t412 = CMC2.*F2.*t2.*t6.*t8.*2.0;
t413 = CMC1.*F1.*t7.*t8.*t17.*2.0;
t414 = F1.*F_11.*t2.*t7.*t8.*2.0;
t415 = CMC1.*F1.*t3.*t8.*t18.*4.0;
t416 = CMC1.*F_11.*t3.*t6.*t8.*2.0;
t417 = CMC1.*F_11.*t6.*t7.*t8.*4.0;
t418 = CMC2.*F2.*t2.*t8.*t18.*4.0;
t419 = CMC2.*F_12.*t2.*t6.*t8.*2.0;
t420 = CMC3.*F3.*t2.*t8.*t17.*2.0;
t421 = CMC3.*F_13.*t2.*t4.*t8.*6.0;
t422 = CMC2.*F2.*t7.*t8.*t19.*2.0;
t423 = CMC3.*F3.*t2.*t8.*t19.*2.0;
t424 = CMC3.*F_13.*t2.*t5.*t8.*2.0;
t425 = F3.*F_13.*t2.*t3.*t8.*4.0;
t426 = CMC3.*F3.*t3.*t8.*t17.*2.0;
t427 = CMC3.*F_13.*t3.*t4.*t8.*2.0;
t428 = F2.*F_12.*t3.*t7.*t8.*2.0;
t429 = CMC2.*F_12.*t6.*t7.*t8.*4.0;
t430 = CMC3.*F3.*t2.*t8.*t18.*2.0;
t431 = CMC3.*F3.*t3.*t8.*t19.*2.0;
t432 = CMC3.*F_13.*t3.*t5.*t8.*6.0;
t433 = CMC3.*F3.*t3.*t8.*t18.*2.0;
t434 = CMC1.*F1.*t6.*t8.*t17.*2.0;
t435 = CMC1.*F_11.*t4.*t6.*t8.*2.0;
t436 = CMC1.*F1.*t5.*t8.*t18.*4.0;
t437 = CMC1.*F1.*t6.*t8.*t19.*4.0;
t438 = CMC1.*F_11.*t5.*t6.*t8.*4.0;
t439 = F1.*F_11.*t3.*t6.*t8.*2.0;
t440 = F1.*F_11.*t5.*t7.*t8.*2.0;
t441 = CMC1.*F1.*t6.*t8.*t18.*4.0;
t442 = CMC2.*F2.*t6.*t8.*t17.*4.0;
t443 = CMC2.*F2.*t4.*t8.*t18.*4.0;
t444 = CMC2.*F_12.*t4.*t6.*t8.*4.0;
t445 = CMC3.*F3.*t4.*t8.*t17.*2.0;
t446 = F2.*F_12.*t2.*t6.*t8.*2.0;
t447 = F3.*F_13.*t2.*t4.*t8.*6.0;
t448 = F1.*F_11.*t6.*t7.*t8.*8.0;
t449 = F2.*F_12.*t4.*t7.*t8.*2.0;
t450 = CMC2.*F2.*t6.*t8.*t19.*2.0;
t451 = CMC2.*F_12.*t5.*t6.*t8.*2.0;
t452 = CMC3.*F3.*t4.*t8.*t19.*2.0;
t453 = CMC3.*F_13.*t4.*t5.*t8.*4.0;
t454 = CMC3.*F3.*t5.*t8.*t17.*2.0;
t455 = F3.*F_13.*t2.*t5.*t8.*2.0;
t456 = F3.*F_13.*t3.*t4.*t8.*2.0;
t457 = CMC2.*F2.*t6.*t8.*t18.*4.0;
t458 = CMC3.*F3.*t4.*t8.*t18.*2.0;
t459 = CMC3.*F_13.*t4.*t6.*t8.*4.0;
t460 = CMC3.*F3.*t5.*t8.*t19.*2.0;
t461 = F3.*F_13.*t3.*t5.*t8.*6.0;
t462 = F2.*F_12.*t6.*t7.*t8.*8.0;
t463 = CMC3.*F3.*t5.*t8.*t18.*2.0;
t464 = CMC3.*F_13.*t5.*t6.*t8.*4.0;
t465 = CMC1.*CMC2.*F1.*F_12.*t13.*6.0;
t466 = CMC1.*CMC2.*F2.*F_11.*t13.*6.0;
t467 = CMC1.*F1.*F2.*F_12.*t13.*2.0;
t468 = CMC2.*F1.*F2.*F_11.*t13.*2.0;
t469 = CMC1.*F2.*F_11.*F_12.*t13.*2.0;
t470 = CMC2.*F1.*F_11.*F_12.*t13.*2.0;
t471 = CMC3.*F1.*F_11.*F_13.*t13.*6.0;
t472 = CMC3.*F2.*F_12.*F_13.*t13.*6.0;
t473 = CMC1.*CMC3.*F1.*F_13.*t20.*2.0;
t474 = CMC1.*CMC3.*F3.*F_11.*t20.*2.0;
t475 = CMC2.*CMC3.*F2.*F_13.*t20.*2.0;
t476 = CMC2.*CMC3.*F3.*F_12.*t20.*2.0;
t477 = CMC1.*F1.*F3.*F_13.*t20.*2.0;
t478 = CMC3.*F1.*F3.*F_11.*t20.*2.0;
t479 = CMC2.*F2.*F3.*F_13.*t20.*2.0;
t480 = CMC3.*F2.*F3.*F_12.*t20.*2.0;
t481 = CMC1.*F3.*F_11.*F_13.*t20.*2.0;
t482 = CMC3.*F1.*F_11.*F_13.*t20.*2.0;
t483 = CMC2.*F3.*F_12.*F_13.*t20.*2.0;
t484 = CMC3.*F2.*F_12.*F_13.*t20.*2.0;
t485 = CMC1.*CMC3.*F3.*F_11.*t3.*t6.*2.0;
t486 = CMC2.*CMC3.*F3.*F_12.*t2.*t6.*2.0;
t487 = CMC1.*CMC2.*F1.*F_12.*t4.*t6.*6.0;
t488 = CMC1.*CMC2.*F2.*F_11.*t5.*t6.*6.0;
t489 = CMC1.*CMC3.*F1.*F3.*t6.*t17.*4.0;
t490 = CMC1.*CMC2.*F1.*F_12.*t3.*t6.*2.0;
t491 = CMC1.*CMC2.*F2.*F_11.*t3.*t6.*2.0;
t492 = CMC1.*CMC2.*F1.*F_12.*t2.*t6.*2.0;
t493 = CMC1.*CMC2.*F2.*F_11.*t2.*t6.*2.0;
t494 = CMC1.*CMC3.*F1.*F3.*t6.*t19.*8.0;
t495 = CMC1.*CMC3.*F3.*F_11.*t5.*t6.*6.0;
t496 = CMC1.*F1.*F3.*F_13.*t3.*t6.*6.0;
t497 = CMC3.*F1.*F3.*F_11.*t3.*t6.*6.0;
t498 = CMC1.*CMC3.*F1.*F3.*t6.*t18.*4.0;
t499 = CMC1.*CMC3.*F1.*F_13.*t4.*t6.*6.0;
t500 = CMC1.*CMC3.*F1.*F_13.*t6.*t7.*2.0;
t501 = CMC2.*CMC3.*F2.*F3.*t6.*t17.*8.0;
t502 = CMC2.*CMC3.*F3.*F_12.*t4.*t6.*6.0;
t503 = CMC2.*F2.*F3.*F_13.*t2.*t6.*6.0;
t504 = CMC3.*F2.*F3.*F_12.*t2.*t6.*6.0;
t505 = CMC1.*CMC3.*F1.*F_13.*t2.*t6.*2.0;
t506 = CMC2.*CMC3.*F2.*F3.*t6.*t19.*4.0;
t507 = CMC2.*CMC3.*F2.*F3.*t6.*t18.*4.0;
t508 = CMC2.*CMC3.*F2.*F_13.*t5.*t6.*6.0;
t509 = CMC2.*CMC3.*F2.*F_13.*t6.*t7.*2.0;
t510 = CMC2.*CMC3.*F2.*F_13.*t3.*t6.*2.0;
t511 = CMC1.*F3.*F_11.*F_13.*t3.*t6.*2.0;
t512 = CMC1.*F3.*F_11.*F_13.*t6.*t7.*6.0;
t513 = CMC2.*F3.*F_12.*F_13.*t2.*t6.*2.0;
t514 = CMC2.*F3.*F_12.*F_13.*t6.*t7.*6.0;
t515 = CMC1.*F1.*F2.*F_12.*t5.*t6.*2.0;
t516 = CMC1.*F1.*F2.*F_12.*t4.*t6.*2.0;
t517 = CMC2.*F1.*F2.*F_11.*t5.*t6.*2.0;
t518 = CMC2.*F1.*F2.*F_11.*t4.*t6.*2.0;
t519 = CMC1.*F1.*F2.*F_12.*t2.*t6.*6.0;
t520 = CMC2.*F1.*F2.*F_11.*t3.*t6.*6.0;
t521 = CMC1.*F1.*F3.*F_13.*t5.*t6.*2.0;
t522 = CMC3.*F1.*F3.*F_11.*t5.*t6.*2.0;
t523 = CMC2.*F2.*F3.*F_13.*t4.*t6.*2.0;
t524 = CMC3.*F2.*F3.*F_12.*t4.*t6.*2.0;
t525 = CMC1.*F3.*F_11.*F_13.*t4.*t6.*6.0;
t526 = CMC1.*F2.*F_11.*F_12.*t5.*t6.*2.0;
t527 = CMC2.*F1.*F_11.*F_12.*t4.*t6.*2.0;
t528 = CMC1.*F2.*F_11.*F_12.*t2.*t6.*2.0;
t529 = CMC2.*F1.*F_11.*F_12.*t3.*t6.*2.0;
t530 = CMC1.*F3.*F_11.*F_13.*t5.*t6.*2.0;
t531 = CMC2.*F3.*F_12.*F_13.*t4.*t6.*2.0;
t532 = CMC3.*F1.*F_11.*F_13.*t4.*t6.*2.0;
t533 = CMC3.*F1.*F_11.*F_13.*t6.*t7.*2.0;
t534 = CMC2.*F3.*F_12.*F_13.*t5.*t6.*6.0;
t535 = CMC3.*F2.*F_12.*F_13.*t5.*t6.*2.0;
t536 = CMC3.*F2.*F_12.*F_13.*t6.*t7.*2.0;
t537 = CMC1.*CMC3.*F1.*F3.*t6.*t8.*4.0;
t538 = CMC1.*CMC3.*F1.*F3.*t4.*t8.*2.0;
t539 = CMC1.*CMC3.*F1.*F3.*t2.*t8.*2.0;
t540 = CMC2.*CMC3.*F2.*F3.*t6.*t8.*4.0;
t541 = CMC2.*CMC3.*F2.*F3.*t5.*t8.*2.0;
t542 = CMC2.*CMC3.*F2.*F3.*t3.*t8.*2.0;
t543 = CMC1.*CMC3.*F_11.*F_13.*t2.*t8.*2.0;
t544 = CMC2.*CMC3.*F_12.*F_13.*t3.*t8.*2.0;
t545 = F1.*F3.*F_11.*F_13.*t6.*t8.*4.0;
t546 = F1.*F3.*F_11.*F_13.*t4.*t8.*2.0;
t547 = F2.*F3.*F_12.*F_13.*t6.*t8.*4.0;
t548 = F2.*F3.*F_12.*F_13.*t5.*t8.*2.0;
t549 = CMC1.*F1.*t3.*t5.*t6.*4.0;
t550 = CMC2.*F2.*t2.*t4.*t6.*4.0;
t551 = CMC1.*F_11.*t3.*t4.*t6.*4.0;
t552 = CMC1.*F_11.*t4.*t6.*t7.*4.0;
t553 = CMC2.*F_12.*t2.*t5.*t6.*4.0;
t554 = CMC2.*F_12.*t5.*t6.*t7.*4.0;
t555 = F1.*F_11.*t2.*t5.*t6.*4.0;
t556 = F2.*F_12.*t3.*t4.*t6.*4.0;
t557 = CMC1.*CMC2.*CMC3.*F1.*F2.*F3.*t6.*1.2e1;
t558 = CMC1.*CMC2.*CMC3.*F3.*F_11.*F_12.*t6.*4.0;
t559 = CMC1.*F1.*F2.*F3.*F_12.*F_13.*t6.*4.0;
t560 = CMC2.*F1.*F2.*F3.*F_11.*F_13.*t6.*4.0;
t561 = CMC3.*F1.*F2.*F3.*F_11.*F_12.*t6.*4.0;
t562 = CMC1.*CMC2.*F1.*F_12.*t6.*t7.*2.0;
t563 = CMC1.*CMC2.*F2.*F_11.*t6.*t7.*2.0;
t564 = CMC1.*CMC3.*F1.*F_13.*t3.*t6.*2.0;
t565 = CMC2.*CMC3.*F2.*F_13.*t2.*t6.*2.0;
t566 = CMC1.*CMC2.*F1.*F2.*t6.*t17.*4.0;
t567 = CMC1.*CMC2.*F1.*F2.*t6.*t19.*4.0;
t568 = CMC1.*CMC2.*F1.*F2.*t6.*t18.*8.0;
t569 = CMC1.*F1.*F2.*F_12.*t6.*t7.*6.0;
t570 = CMC2.*F1.*F2.*F_11.*t6.*t7.*6.0;
t571 = CMC1.*CMC3.*F1.*F_13.*t5.*t6.*6.0;
t572 = CMC2.*CMC3.*F2.*F_13.*t4.*t6.*6.0;
t573 = CMC2.*F1.*F_11.*F_12.*t2.*t6.*6.0;
t574 = CMC1.*F2.*F_11.*F_12.*t3.*t6.*6.0;
t575 = CMC1.*F2.*F_11.*F_12.*t6.*t7.*2.0;
t576 = CMC2.*F1.*F_11.*F_12.*t6.*t7.*2.0;
t577 = CMC3.*F1.*F_11.*F_13.*t2.*t6.*6.0;
t578 = CMC3.*F1.*F_11.*F_13.*t3.*t6.*2.0;
t579 = CMC3.*F2.*F_12.*F_13.*t2.*t6.*2.0;
t580 = CMC3.*F2.*F_12.*F_13.*t3.*t6.*6.0;
t581 = CMC1.*F2.*F_11.*F_12.*t4.*t6.*6.0;
t582 = CMC2.*F1.*F_11.*F_12.*t5.*t6.*6.0;
t583 = CMC3.*F1.*F_11.*F_13.*t5.*t6.*2.0;
t584 = CMC3.*F2.*F_12.*F_13.*t4.*t6.*2.0;
t585 = CMC1.*CMC3.*F1.*F3.*t3.*t8.*2.0;
t586 = CMC2.*CMC3.*F2.*F3.*t2.*t8.*2.0;
t587 = CMC1.*CMC2.*F1.*F_12.*t7.*t8.*2.0;
t588 = CMC1.*CMC2.*F2.*F_11.*t7.*t8.*2.0;
t589 = CMC1.*CMC3.*F_11.*F_13.*t3.*t8.*2.0;
t590 = CMC2.*CMC3.*F_12.*F_13.*t2.*t8.*2.0;
t591 = CMC1.*CMC2.*F1.*F2.*t6.*t8.*2.0;
t592 = CMC1.*CMC3.*F1.*F3.*t5.*t8.*2.0;
t593 = CMC2.*CMC3.*F2.*F3.*t4.*t8.*2.0;
t594 = CMC1.*CMC3.*F3.*F_11.*t4.*t8.*2.0;
t595 = CMC3.*F1.*F3.*F_11.*t2.*t8.*2.0;
t596 = CMC1.*F1.*F3.*F_13.*t7.*t8.*4.0;
t597 = CMC2.*CMC3.*F3.*F_12.*t5.*t8.*2.0;
t598 = CMC3.*F2.*F3.*F_12.*t3.*t8.*2.0;
t599 = CMC2.*F2.*F3.*F_13.*t7.*t8.*4.0;
t600 = CMC1.*CMC2.*F_11.*F_12.*t6.*t8.*2.0;
t601 = CMC1.*CMC3.*F_11.*F_13.*t4.*t8.*6.0;
t602 = CMC1.*F2.*F_11.*F_12.*t7.*t8.*2.0;
t603 = CMC2.*F1.*F_11.*F_12.*t7.*t8.*2.0;
t604 = CMC1.*CMC3.*F_11.*F_13.*t5.*t8.*2.0;
t605 = CMC1.*CMC3.*F_11.*F_13.*t6.*t8.*8.0;
t606 = CMC2.*CMC3.*F_12.*F_13.*t4.*t8.*2.0;
t607 = CMC2.*CMC3.*F_12.*F_13.*t5.*t8.*6.0;
t608 = CMC2.*CMC3.*F_12.*F_13.*t6.*t8.*8.0;
t609 = F1.*F3.*F_11.*F_13.*t2.*t8.*6.0;
t610 = F1.*F3.*F_11.*F_13.*t3.*t8.*2.0;
t611 = F2.*F3.*F_12.*F_13.*t2.*t8.*2.0;
t612 = F1.*F3.*F_11.*F_13.*t7.*t8.*4.0;
t613 = F2.*F3.*F_12.*F_13.*t3.*t8.*6.0;
t614 = F2.*F3.*F_12.*F_13.*t7.*t8.*4.0;
t615 = F1.*F2.*F_11.*F_12.*t6.*t8.*2.0;
t616 = F1.*F3.*F_11.*F_13.*t5.*t8.*2.0;
t617 = F2.*F3.*F_12.*F_13.*t4.*t8.*2.0;
t618 = CMC1.*CMC2.*CMC3.*F1.*F_12.*F_13.*t6.*4.0;
t619 = CMC1.*CMC2.*CMC3.*F2.*F_11.*F_13.*t6.*4.0;
t620 = CMC1.*CMC2.*CMC3.*F1.*F2.*F_13.*t8.*8.0;
t621 = CMC1.*CMC2.*CMC3.*F1.*F3.*F_12.*t8.*4.0;
t622 = CMC1.*CMC2.*CMC3.*F2.*F3.*F_11.*t8.*4.0;
t623 = CMC1.*CMC2.*F1.*F2.*F3.*F_13.*t8.*8.0;
t624 = CMC1.*CMC3.*F1.*F2.*F3.*F_12.*t8.*4.0;
t625 = CMC2.*CMC3.*F1.*F2.*F3.*F_11.*t8.*4.0;
t626 = CMC1.*CMC2.*F1.*F3.*F_12.*F_13.*t8.*4.0;
t627 = CMC1.*CMC2.*F2.*F3.*F_11.*F_13.*t8.*4.0;
t628 = CMC1.*CMC3.*F1.*F2.*F_12.*F_13.*t8.*4.0;
t629 = CMC2.*CMC3.*F1.*F2.*F_11.*F_13.*t8.*4.0;
t843 = CMC3.*F3.*t4.*t6.*t7.*2.0;
t844 = CMC3.*F3.*t5.*t6.*t7.*2.0;
t845 = CMC3.*F3.*t6.*t7.*t17.*4.0;
t846 = CMC3.*F3.*t6.*t7.*t19.*4.0;
t847 = t2.*t8.*t13.*2.0;
t848 = t6.*t8.*t11;
t849 = t7.*t8.*t12;
t850 = t3.*t8.*t13.*2.0;
t851 = t7.*t8.*t14;
t852 = t6.*t8.*t15;
t853 = t8.*t11.*t18;
t854 = t8.*t15.*t18;
t855 = t8.*t12.*t18;
t856 = t8.*t13.*t17.*2.0;
t857 = t8.*t14.*t18;
t858 = t8.*t13.*t19.*2.0;
t859 = CMC1.*F_11.*t6.*t13.*2.0;
t860 = CMC2.*F_12.*t6.*t13.*2.0;
t861 = CMC3.*F3.*t2.*t13.*2.0;
t862 = CMC3.*F3.*t3.*t13.*2.0;
t863 = CMC1.*F1.*t2.*t13.*2.0;
t864 = CMC2.*F2.*t3.*t13.*2.0;
t865 = CMC1.*F_11.*t2.*t13.*2.0;
t866 = CMC3.*F3.*t13.*t17.*4.0;
t867 = F3.*F_13.*t2.*t13.*2.0;
t868 = F3.*F_13.*t6.*t11.*2.0;
t869 = CMC2.*F_12.*t3.*t13.*2.0;
t870 = CMC3.*F3.*t13.*t19.*4.0;
t871 = F3.*F_13.*t3.*t13.*2.0;
t872 = F3.*F_13.*t6.*t15.*2.0;
t873 = t2.*t4.*t7.*t8;
t874 = t2.*t3.*t6.*t8.*2.0;
t875 = t3.*t5.*t7.*t8;
t876 = t2.*t7.*t8.*t17;
t877 = t2.*t3.*t8.*t18.*2.0;
t878 = t3.*t7.*t8.*t19;
t879 = t2.*t4.*t6.*t8;
t880 = t2.*t5.*t6.*t8.*2.0;
t881 = t3.*t4.*t6.*t8.*2.0;
t882 = t4.*t5.*t7.*t8.*2.0;
t883 = t3.*t5.*t6.*t8;
t884 = t4.*t6.*t7.*t8.*2.0;
t885 = t5.*t6.*t7.*t8.*2.0;
t886 = t2.*t4.*t8.*t18.*6.0;
t887 = t2.*t6.*t8.*t17;
t888 = t4.*t7.*t8.*t17;
t889 = t2.*t5.*t8.*t18.*2.0;
t890 = t2.*t6.*t8.*t19.*2.0;
t891 = t3.*t4.*t8.*t18.*2.0;
t892 = t3.*t6.*t8.*t17.*2.0;
t893 = t2.*t6.*t8.*t18.*2.0;
t894 = t3.*t5.*t8.*t18.*6.0;
t895 = t3.*t6.*t8.*t19;
t896 = t5.*t7.*t8.*t19;
t897 = t6.*t7.*t8.*t17.*6.0;
t898 = t3.*t6.*t8.*t18.*2.0;
t899 = t6.*t7.*t8.*t19.*6.0;
t900 = t4.*t6.*t8.*t17;
t901 = t4.*t5.*t8.*t18.*2.0;
t902 = t4.*t6.*t8.*t19.*2.0;
t903 = t5.*t6.*t8.*t17.*2.0;
t904 = t4.*t6.*t8.*t18.*2.0;
t905 = t5.*t6.*t8.*t19;
t906 = t5.*t6.*t8.*t18.*2.0;
t907 = CMC1.*F1.*t3.*t13.*2.0;
t908 = CMC1.*CMC3.*F1.*F3.*t4.*t6.*2.0;
t909 = CMC1.*CMC3.*F1.*F3.*t6.*t7.*2.0;
t910 = CMC2.*F2.*t2.*t13.*2.0;
t911 = CMC1.*CMC3.*F1.*F3.*t2.*t6.*2.0;
t912 = CMC2.*CMC3.*F2.*F3.*t5.*t6.*2.0;
t913 = CMC2.*CMC3.*F2.*F3.*t6.*t7.*2.0;
t914 = CMC2.*CMC3.*F2.*F3.*t3.*t6.*2.0;
t915 = CMC1.*F_11.*t3.*t13.*2.0;
t916 = CMC1.*F_11.*t7.*t13.*6.0;
t917 = CMC2.*F_12.*t2.*t13.*2.0;
t918 = CMC2.*F_12.*t7.*t13.*6.0;
t919 = CMC1.*F1.*t13.*t17.*2.0;
t920 = CMC1.*F_11.*t4.*t13.*2.0;
t921 = CMC1.*F1.*t13.*t19.*4.0;
t922 = CMC1.*F_11.*t5.*t13.*4.0;
t923 = CMC1.*F_11.*t6.*t14.*2.0;
t924 = F1.*F_11.*t3.*t13.*2.0;
t925 = F1.*F_11.*t6.*t15.*2.0;
t926 = CMC1.*F1.*t13.*t18.*2.0;
t927 = CMC2.*F2.*t13.*t17.*4.0;
t928 = CMC2.*F_12.*t4.*t13.*4.0;
t929 = CMC2.*F_12.*t6.*t12.*2.0;
t930 = F2.*F_12.*t2.*t13.*2.0;
t931 = F2.*F_12.*t6.*t11.*2.0;
t932 = F1.*F_11.*t7.*t13.*6.0;
t933 = F1.*F_11.*t6.*t16.*2.0;
t934 = CMC2.*F2.*t13.*t19.*2.0;
t935 = CMC2.*F_12.*t5.*t13.*2.0;
t936 = CMC2.*F2.*t13.*t18.*2.0;
t937 = CMC3.*F_13.*t4.*t13.*2.0;
t938 = CMC3.*F_13.*t6.*t12.*2.0;
t939 = F2.*F_12.*t7.*t13.*6.0;
t940 = F2.*F_12.*t6.*t16.*2.0;
t941 = CMC3.*F_13.*t5.*t13.*2.0;
t942 = CMC3.*F_13.*t6.*t14.*2.0;
t943 = F1.*F3.*F_11.*F_13.*t4.*t6.*2.0;
t944 = F2.*F3.*F_12.*F_13.*t5.*t6.*2.0;
t945 = CMC1.*F1.*t18.*t20.*2.0;
t946 = CMC1.*F_11.*t6.*t20.*2.0;
t947 = F1.*F_11.*t7.*t20.*2.0;
t948 = CMC2.*F2.*t18.*t20.*2.0;
t949 = CMC2.*F_12.*t6.*t20.*2.0;
t950 = CMC3.*F3.*t17.*t20.*2.0;
t951 = CMC3.*F_13.*t4.*t20.*2.0;
t952 = F3.*F_13.*t2.*t20.*2.0;
t953 = F2.*F_12.*t7.*t20.*2.0;
t954 = CMC3.*F3.*t19.*t20.*2.0;
t955 = CMC3.*F_13.*t5.*t20.*2.0;
t956 = F3.*F_13.*t3.*t20.*2.0;
t957 = CMC1.*F1.*t3.*t4.*t6.*2.0;
t958 = CMC1.*F1.*t4.*t6.*t7.*2.0;
t959 = CMC2.*F2.*t2.*t5.*t6.*2.0;
t960 = CMC3.*F3.*t2.*t5.*t6.*2.0;
t961 = CMC3.*F3.*t3.*t4.*t6.*2.0;
t962 = CMC2.*F2.*t5.*t6.*t7.*2.0;
t963 = CMC3.*F3.*t2.*t6.*t17.*2.0;
t964 = CMC3.*F3.*t2.*t6.*t19.*4.0;
t965 = F3.*F_13.*t2.*t3.*t6.*4.0;
t966 = CMC3.*F3.*t3.*t6.*t17.*4.0;
t967 = CMC3.*F3.*t2.*t6.*t18.*2.0;
t968 = F3.*F_13.*t2.*t6.*t7.*2.0;
t969 = CMC3.*F3.*t3.*t6.*t19.*2.0;
t970 = CMC3.*F3.*t3.*t6.*t18.*2.0;
t971 = F3.*F_13.*t3.*t6.*t7.*2.0;
t972 = CMC1.*F1.*t2.*t5.*t6.*2.0;
t973 = CMC2.*F2.*t3.*t4.*t6.*2.0;
t974 = CMC1.*F1.*t4.*t6.*t19.*4.0;
t975 = CMC1.*F1.*t2.*t6.*t19.*4.0;
t976 = CMC1.*F_11.*t2.*t5.*t6.*2.0;
t977 = F1.*F_11.*t3.*t4.*t6.*2.0;
t978 = CMC1.*F1.*t4.*t6.*t18.*4.0;
t979 = CMC2.*F2.*t5.*t6.*t17.*4.0;
t980 = CMC3.*F3.*t4.*t6.*t17.*2.0;
t981 = F3.*F_13.*t2.*t4.*t6.*6.0;
t982 = F2.*F_12.*t2.*t5.*t6.*2.0;
t983 = CMC1.*F1.*t2.*t6.*t18.*4.0;
t984 = CMC2.*F2.*t3.*t6.*t17.*4.0;
t985 = CMC2.*F_12.*t3.*t4.*t6.*2.0;
t986 = F1.*F_11.*t4.*t6.*t7.*2.0;
t987 = CMC3.*F3.*t4.*t6.*t19.*4.0;
t988 = CMC3.*F3.*t5.*t6.*t17.*4.0;
t989 = F3.*F_13.*t2.*t5.*t6.*2.0;
t990 = F3.*F_13.*t3.*t4.*t6.*2.0;
t991 = CMC2.*F2.*t5.*t6.*t18.*4.0;
t992 = CMC3.*F3.*t4.*t6.*t18.*2.0;
t993 = CMC3.*F3.*t5.*t6.*t19.*2.0;
t994 = F3.*F_13.*t3.*t5.*t6.*6.0;
t995 = CMC2.*F2.*t3.*t6.*t18.*4.0;
t996 = F2.*F_12.*t5.*t6.*t7.*2.0;
t997 = CMC3.*F_13.*t4.*t6.*t7.*2.0;
t998 = CMC3.*F3.*t5.*t6.*t18.*2.0;
t999 = CMC3.*F_13.*t5.*t6.*t7.*2.0;
t1000 = CMC1.*CMC3.*F1.*F3.*t13.*2.0;
t1001 = CMC2.*CMC3.*F2.*F3.*t13.*2.0;
t1002 = F1.*F3.*F_11.*F_13.*t13.*2.0;
t1003 = F2.*F3.*F_12.*F_13.*t13.*2.0;
t1004 = CMC1.*F1.*t6.*t7.*t8.*4.0;
t1005 = CMC3.*F3.*t2.*t4.*t8.*4.0;
t1006 = CMC2.*F2.*t6.*t7.*t8.*4.0;
t1007 = CMC3.*F3.*t3.*t5.*t8.*4.0;
t1008 = CMC1.*F_11.*t4.*t7.*t8.*4.0;
t1009 = CMC1.*F_11.*t5.*t7.*t8.*2.0;
t1010 = CMC2.*F_12.*t4.*t7.*t8.*2.0;
t1011 = CMC2.*F_12.*t5.*t7.*t8.*4.0;
t1012 = CMC3.*F_13.*t2.*t6.*t8.*4.0;
t1013 = CMC3.*F_13.*t3.*t6.*t8.*4.0;
t1014 = F1.*F_11.*t2.*t6.*t8.*4.0;
t1015 = F2.*F_12.*t3.*t6.*t8.*4.0;
t1016 = F3.*F_13.*t4.*t7.*t8.*4.0;
t1017 = F3.*F_13.*t5.*t7.*t8.*4.0;
t1018 = CMC1.*CMC2.*F1.*F2.*t13.*2.0;
t1019 = CMC1.*CMC3.*F1.*F_13.*t13.*2.0;
t1020 = CMC2.*CMC3.*F2.*F_13.*t13.*2.0;
t1021 = CMC1.*CMC2.*F_11.*F_12.*t13.*2.0;
t1022 = CMC1.*CMC3.*F_11.*F_13.*t13.*6.0;
t1023 = CMC2.*CMC3.*F_12.*F_13.*t13.*6.0;
t1024 = F1.*F2.*F_11.*F_12.*t13.*2.0;
t1025 = CMC1.*CMC3.*F1.*F3.*t20.*2.0;
t1026 = CMC2.*CMC3.*F2.*F3.*t20.*2.0;
t1027 = CMC1.*CMC3.*F_11.*F_13.*t20.*2.0;
t1028 = CMC2.*CMC3.*F_12.*F_13.*t20.*2.0;
t1029 = F1.*F3.*F_11.*F_13.*t20.*2.0;
t1030 = F2.*F3.*F_12.*F_13.*t20.*2.0;
t1031 = CMC1.*CMC3.*F1.*F3.*t3.*t6.*2.0;
t1032 = CMC2.*CMC3.*F2.*F3.*t2.*t6.*2.0;
t1033 = CMC1.*CMC2.*F1.*F2.*t5.*t6.*2.0;
t1034 = CMC1.*CMC2.*F1.*F2.*t4.*t6.*2.0;
t1035 = CMC1.*CMC2.*F1.*F2.*t3.*t6.*2.0;
t1036 = CMC1.*CMC2.*F1.*F2.*t2.*t6.*2.0;
t1037 = CMC1.*CMC3.*F1.*F3.*t5.*t6.*2.0;
t1038 = CMC2.*CMC3.*F2.*F3.*t4.*t6.*2.0;
t1039 = CMC1.*CMC3.*F3.*F_11.*t4.*t6.*2.0;
t1040 = CMC3.*F1.*F3.*F_11.*t2.*t6.*2.0;
t1041 = CMC1.*F1.*F3.*F_13.*t6.*t7.*2.0;
t1042 = CMC2.*CMC3.*F3.*F_12.*t5.*t6.*2.0;
t1043 = CMC3.*F2.*F3.*F_12.*t3.*t6.*2.0;
t1044 = CMC2.*F2.*F3.*F_13.*t6.*t7.*2.0;
t1045 = CMC1.*CMC2.*F_11.*F_12.*t3.*t6.*2.0;
t1046 = CMC1.*CMC2.*F_11.*F_12.*t2.*t6.*2.0;
t1047 = CMC1.*CMC3.*F_11.*F_13.*t6.*t7.*2.0;
t1048 = CMC1.*CMC3.*F_11.*F_13.*t2.*t6.*2.0;
t1049 = CMC2.*CMC3.*F_12.*F_13.*t6.*t7.*2.0;
t1050 = CMC2.*CMC3.*F_12.*F_13.*t3.*t6.*2.0;
t1051 = F1.*F3.*F_11.*F_13.*t2.*t6.*6.0;
t1052 = F1.*F3.*F_11.*F_13.*t3.*t6.*2.0;
t1053 = F2.*F3.*F_12.*F_13.*t2.*t6.*2.0;
t1054 = F1.*F3.*F_11.*F_13.*t6.*t7.*6.0;
t1055 = F2.*F3.*F_12.*F_13.*t3.*t6.*6.0;
t1056 = F2.*F3.*F_12.*F_13.*t6.*t7.*6.0;
t1057 = F1.*F2.*F_11.*F_12.*t5.*t6.*2.0;
t1058 = F1.*F2.*F_11.*F_12.*t4.*t6.*2.0;
t1059 = F1.*F3.*F_11.*F_13.*t5.*t6.*2.0;
t1060 = F2.*F3.*F_12.*F_13.*t4.*t6.*2.0;
t1061 = CMC1.*CMC3.*F1.*F_13.*t4.*t8.*6.0;
t1062 = CMC1.*CMC3.*F3.*F_11.*t6.*t8.*8.0;
t1063 = CMC1.*CMC3.*F1.*F_13.*t2.*t8.*2.0;
t1064 = CMC1.*CMC3.*F3.*F_11.*t2.*t8.*2.0;
t1065 = CMC2.*CMC3.*F2.*F_13.*t5.*t8.*6.0;
t1066 = CMC2.*CMC3.*F3.*F_12.*t6.*t8.*8.0;
t1067 = CMC2.*CMC3.*F2.*F_13.*t3.*t8.*2.0;
t1068 = CMC2.*CMC3.*F3.*F_12.*t3.*t8.*2.0;
t1069 = CMC1.*F1.*F3.*F_13.*t6.*t8.*4.0;
t1070 = CMC1.*F1.*F3.*F_13.*t4.*t8.*2.0;
t1071 = CMC3.*F1.*F3.*F_11.*t6.*t8.*4.0;
t1072 = CMC3.*F1.*F3.*F_11.*t4.*t8.*2.0;
t1073 = CMC1.*F1.*F3.*F_13.*t2.*t8.*6.0;
t1074 = CMC3.*F1.*F3.*F_11.*t7.*t8.*4.0;
t1075 = CMC2.*F2.*F3.*F_13.*t6.*t8.*4.0;
t1076 = CMC2.*F2.*F3.*F_13.*t5.*t8.*2.0;
t1077 = CMC3.*F2.*F3.*F_12.*t6.*t8.*4.0;
t1078 = CMC3.*F2.*F3.*F_12.*t5.*t8.*2.0;
t1079 = CMC2.*F2.*F3.*F_13.*t3.*t8.*6.0;
t1080 = CMC3.*F2.*F3.*F_12.*t7.*t8.*4.0;
t1081 = CMC1.*F3.*F_11.*F_13.*t6.*t8.*4.0;
t1082 = CMC3.*F1.*F_11.*F_13.*t4.*t8.*2.0;
t1083 = CMC1.*F3.*F_11.*F_13.*t2.*t8.*2.0;
t1084 = CMC2.*F3.*F_12.*F_13.*t6.*t8.*4.0;
t1085 = CMC3.*F2.*F_12.*F_13.*t5.*t8.*2.0;
t1086 = CMC2.*F3.*F_12.*F_13.*t3.*t8.*2.0;
t1087 = CMC1.*F1.*t5.*t6.*t7.*2.0;
t1088 = CMC2.*F2.*t4.*t6.*t7.*2.0;
t1089 = CMC1.*F1.*t3.*t6.*t17.*2.0;
t1090 = F1.*F_11.*t2.*t3.*t6.*2.0;
t1091 = CMC1.*F1.*t3.*t6.*t19.*2.0;
t1092 = CMC1.*F_11.*t3.*t5.*t6.*6.0;
t1093 = CMC1.*F1.*t6.*t7.*t17.*2.0;
t1094 = CMC2.*F2.*t2.*t6.*t17.*2.0;
t1095 = CMC2.*F_12.*t2.*t4.*t6.*6.0;
t1096 = F1.*F_11.*t2.*t6.*t7.*2.0;
t1097 = CMC1.*F1.*t3.*t6.*t18.*4.0;
t1098 = CMC1.*F1.*t6.*t7.*t19.*4.0;
t1099 = CMC1.*F_11.*t5.*t6.*t7.*2.0;
t1100 = CMC2.*F2.*t2.*t6.*t19.*2.0;
t1101 = F2.*F_12.*t2.*t3.*t6.*2.0;
t1102 = F1.*F_11.*t3.*t6.*t7.*4.0;
t1103 = CMC1.*F1.*t6.*t7.*t18.*2.0;
t1104 = CMC2.*F2.*t6.*t7.*t17.*4.0;
t1105 = CMC2.*F_12.*t4.*t6.*t7.*2.0;
t1106 = CMC2.*F2.*t2.*t6.*t18.*4.0;
t1107 = CMC3.*F_13.*t2.*t4.*t6.*6.0;
t1108 = F2.*F_12.*t2.*t6.*t7.*4.0;
t1109 = CMC2.*F2.*t6.*t7.*t19.*2.0;
t1110 = CMC3.*F_13.*t2.*t5.*t6.*2.0;
t1111 = CMC3.*F_13.*t3.*t4.*t6.*2.0;
t1112 = F2.*F_12.*t3.*t6.*t7.*2.0;
t1113 = CMC2.*F2.*t6.*t7.*t18.*2.0;
t1114 = CMC3.*F_13.*t3.*t5.*t6.*6.0;
t1115 = CMC1.*F1.*t5.*t6.*t17.*2.0;
t1116 = CMC1.*F_11.*t4.*t5.*t6.*2.0;
t1117 = CMC1.*F1.*t5.*t6.*t19.*2.0;
t1118 = CMC2.*F2.*t4.*t6.*t17.*2.0;
t1119 = F2.*F_12.*t2.*t4.*t6.*6.0;
t1120 = F1.*F_11.*t3.*t5.*t6.*6.0;
t1121 = CMC1.*F1.*t5.*t6.*t18.*4.0;
t1122 = CMC2.*F2.*t4.*t6.*t19.*2.0;
t1123 = CMC2.*F_12.*t4.*t5.*t6.*2.0;
t1124 = F1.*F_11.*t5.*t6.*t7.*2.0;
t1125 = CMC2.*F2.*t4.*t6.*t18.*4.0;
t1126 = F2.*F_12.*t4.*t6.*t7.*2.0;
t1127 = CMC3.*F_13.*t4.*t5.*t6.*4.0;
t1128 = CMC1.*CMC2.*CMC3.*F1.*F3.*F_12.*t6.*8.0;
t1129 = CMC1.*CMC2.*CMC3.*F2.*F3.*F_11.*t6.*8.0;
t1130 = CMC1.*CMC2.*F1.*F2.*F3.*F_13.*t6.*8.0;
t1131 = CMC1.*CMC3.*F1.*F2.*F3.*F_12.*t6.*8.0;
t1132 = CMC2.*CMC3.*F1.*F2.*F3.*F_11.*t6.*8.0;
t1133 = CMC1.*CMC2.*F1.*F3.*F_12.*F_13.*t6.*4.0;
t1134 = CMC1.*CMC2.*F2.*F3.*F_11.*F_13.*t6.*4.0;
t1135 = CMC1.*CMC3.*F2.*F3.*F_11.*F_12.*t6.*4.0;
t1136 = CMC2.*CMC3.*F1.*F3.*F_11.*F_12.*t6.*4.0;
t1137 = CMC1.*CMC2.*F1.*F2.*t6.*t7.*2.0;
t1138 = CMC1.*CMC2.*F_11.*F_12.*t6.*t7.*2.0;
t1139 = CMC1.*CMC3.*F_11.*F_13.*t3.*t6.*2.0;
t1140 = CMC2.*CMC3.*F_12.*F_13.*t2.*t6.*2.0;
t1141 = CMC1.*CMC2.*F2.*F_11.*t4.*t6.*2.0;
t1142 = CMC2.*F1.*F2.*F_11.*t2.*t6.*2.0;
t1143 = CMC1.*CMC2.*F1.*F_12.*t5.*t6.*2.0;
t1144 = CMC1.*F1.*F2.*F_12.*t3.*t6.*2.0;
t1145 = CMC1.*CMC2.*F_11.*F_12.*t4.*t6.*6.0;
t1146 = CMC1.*CMC2.*F_11.*F_12.*t5.*t6.*6.0;
t1147 = CMC1.*CMC3.*F_11.*F_13.*t4.*t6.*6.0;
t1148 = CMC1.*CMC3.*F_11.*F_13.*t5.*t6.*2.0;
t1149 = CMC2.*CMC3.*F_12.*F_13.*t4.*t6.*2.0;
t1150 = CMC2.*CMC3.*F_12.*F_13.*t5.*t6.*6.0;
t1151 = F1.*F2.*F_11.*F_12.*t2.*t6.*6.0;
t1152 = F1.*F2.*F_11.*F_12.*t3.*t6.*6.0;
t1153 = F1.*F2.*F_11.*F_12.*t6.*t7.*2.0;
t1154 = CMC1.*CMC2.*F1.*F2.*t7.*t8.*2.0;
t1155 = CMC1.*CMC3.*F1.*F_13.*t3.*t8.*2.0;
t1156 = CMC1.*CMC3.*F3.*F_11.*t3.*t8.*2.0;
t1157 = CMC2.*CMC3.*F2.*F_13.*t2.*t8.*2.0;
t1158 = CMC2.*CMC3.*F3.*F_12.*t2.*t8.*2.0;
t1159 = CMC1.*CMC2.*F_11.*F_12.*t7.*t8.*2.0;
t1160 = CMC1.*CMC2.*F1.*F2.*t8.*t18.*8.0;
t1161 = CMC1.*CMC2.*F1.*F_12.*t6.*t8.*6.0;
t1162 = CMC1.*CMC2.*F2.*F_11.*t6.*t8.*6.0;
t1163 = CMC1.*CMC3.*F1.*F3.*t8.*t17.*4.0;
t1164 = CMC1.*F1.*F2.*F_12.*t7.*t8.*2.0;
t1165 = CMC2.*F1.*F2.*F_11.*t7.*t8.*2.0;
t1166 = CMC1.*CMC3.*F1.*F3.*t8.*t19.*4.0;
t1167 = CMC1.*CMC3.*F1.*F_13.*t5.*t8.*6.0;
t1168 = CMC1.*CMC3.*F3.*F_11.*t5.*t8.*2.0;
t1169 = CMC1.*F1.*F3.*F_13.*t3.*t8.*6.0;
t1170 = CMC3.*F1.*F3.*F_11.*t3.*t8.*2.0;
t1171 = CMC1.*CMC3.*F1.*F3.*t8.*t18.*4.0;
t1172 = CMC2.*CMC3.*F2.*F3.*t8.*t17.*4.0;
t1173 = CMC2.*CMC3.*F2.*F_13.*t4.*t8.*6.0;
t1174 = CMC2.*CMC3.*F3.*F_12.*t4.*t8.*2.0;
t1175 = CMC2.*F2.*F3.*F_13.*t2.*t8.*6.0;
t1176 = CMC3.*F2.*F3.*F_12.*t2.*t8.*2.0;
t1177 = CMC2.*CMC3.*F2.*F3.*t8.*t19.*4.0;
t1178 = CMC2.*CMC3.*F2.*F3.*t8.*t18.*4.0;
t1179 = CMC3.*F1.*F_11.*F_13.*t2.*t8.*6.0;
t1180 = CMC1.*F3.*F_11.*F_13.*t3.*t8.*2.0;
t1181 = CMC3.*F1.*F_11.*F_13.*t3.*t8.*2.0;
t1182 = CMC1.*F3.*F_11.*F_13.*t7.*t8.*4.0;
t1183 = CMC2.*F3.*F_12.*F_13.*t2.*t8.*2.0;
t1184 = CMC3.*F2.*F_12.*F_13.*t2.*t8.*2.0;
t1185 = CMC3.*F2.*F_12.*F_13.*t3.*t8.*6.0;
t1186 = CMC2.*F3.*F_12.*F_13.*t7.*t8.*4.0;
t1187 = CMC1.*F1.*F2.*F_12.*t6.*t8.*2.0;
t1188 = CMC2.*F1.*F2.*F_11.*t6.*t8.*2.0;
t1189 = CMC1.*F1.*F3.*F_13.*t5.*t8.*2.0;
t1190 = CMC3.*F1.*F3.*F_11.*t5.*t8.*2.0;
t1191 = CMC2.*F2.*F3.*F_13.*t4.*t8.*2.0;
t1192 = CMC3.*F2.*F3.*F_12.*t4.*t8.*2.0;
t1193 = CMC1.*F2.*F_11.*F_12.*t6.*t8.*2.0;
t1194 = CMC1.*F3.*F_11.*F_13.*t4.*t8.*6.0;
t1195 = CMC2.*F1.*F_11.*F_12.*t6.*t8.*2.0;
t1196 = F1.*F2.*F_11.*F_12.*t7.*t8.*2.0;
t1197 = CMC1.*F3.*F_11.*F_13.*t5.*t8.*2.0;
t1198 = CMC3.*F1.*F_11.*F_13.*t5.*t8.*2.0;
t1199 = CMC2.*F3.*F_12.*F_13.*t4.*t8.*2.0;
t1200 = CMC3.*F1.*F_11.*F_13.*t6.*t8.*8.0;
t1201 = CMC3.*F2.*F_12.*F_13.*t4.*t8.*2.0;
t1202 = CMC2.*F3.*F_12.*F_13.*t5.*t8.*6.0;
t1203 = CMC3.*F2.*F_12.*F_13.*t6.*t8.*8.0;
t1204 = CMC1.*CMC2.*CMC3.*F1.*F2.*F_13.*t6.*8.0;
t1205 = CMC1.*CMC3.*F1.*F2.*F_12.*F_13.*t6.*4.0;
t1206 = CMC2.*CMC3.*F1.*F2.*F_11.*F_13.*t6.*4.0;
t1207 = CMC1.*CMC2.*CMC3.*F1.*F2.*F3.*t8.*8.0;
t1208 = CMC1.*CMC2.*CMC3.*F1.*F_12.*F_13.*t8.*4.0;
t1209 = CMC1.*CMC2.*CMC3.*F2.*F_11.*F_13.*t8.*4.0;
t1210 = CMC1.*F1.*F2.*F3.*F_12.*F_13.*t8.*4.0;
t1211 = CMC2.*F1.*F2.*F3.*F_11.*F_13.*t8.*4.0;
t630 = t253+t254+t255+t256+t257+t258+t259+t260+t261+t262+t263+t264+t265+t266+t267+t268+t269+t270+t271+t272+t273+t274+t275+t276+t277+t278+t279+t280+t281+t282+t283+t284+t285+t286+t287+t288+t289+t290+t291+t292+t293+t294+t295+t296+t297+t298+t299+t300+t301+t302+t303+t304+t305+t306+t307+t308+t309+t310+t311+t312+t313+t314+t315+t316+t317+t318+t319+t320+t321+t322+t323+t324+t325+t326+t327+t328+t329+t330+t331+t332+t333+t334+t335+t336+t337+t338+t339+t340+t341+t342+t343+t344+t345+t346+t347+t348+t349+t350+t351+t352+t353+t354+t355+t356+t357+t358+t359+t360+t361+t362+t363+t364+t365+t366+t367+t368+t369+t370+t371+t372+t373+t374+t375+t376+t377+t378+t379+t380+t381+t382+t383+t384+t385+t386+t387+t388+t389+t390+t391+t392+t393+t394+t395+t396+t397+t398+t399+t400+t401+t402+t403+t404+t405+t406+t407+t408+t409+t410+t411+t412+t413+t414+t415+t416+t417+t418+t419+t420+t421+t422+t423+t424+t425+t426+t427+t428+t429+t430+t431+t432+t433+t434+t435+t436+t437+t438+t439+t440+t441+t442+t443+t444+t445+t446+t447+t448+t449+t450+t451+t452+t453+t454+t455+t456+t457+t458+t459+t460+t461+t462+t463+t464+t465+t466+t467+t468+t469+t470+t471+t472+t473+t474+t475+t476+t477+t478+t479+t480+t481+t482+t483+t484+t485+t486+t487+t488+t489+t490+t491+t492+t493+t494+t495+t496+t497+t498+t499+t500+t501+t502+t503+t504+t505+t506+t507+t508+t509+t510+t511+t512+t513+t514+t515+t516+t517+t518+t519+t520+t521+t522+t523+t524+t525+t526+t527+t528+t529+t530+t531+t532+t533+t534+t535+t536+t537+t538+t539+t540+t541+t542+t543+t544+t545+t546+t547+t548+t549+t550+t551+t552+t553+t554+t555+t556+t557+t558+t559+t560+t561+t562+t563+t564+t565+t566+t567+t568+t569+t570+t571+t572+t573+t574+t575+t576+t577+t578+t579+t580+t581+t582+t583+t584+t585+t586+t587+t588+t589+t590+t591+t592+t593+t594+t595+t596+t597+t598+t599+t600+t601+t602+t603+t604+t605+t606+t607+t608+t609+t610+t611+t612+t613+t614+t615+t616+t617+t618+t619+t620+t621+t622+t623+t624+t625+t626+t627+t628+t629-t843-t844-t845-t846-t847-t848-t849-t850-t851-t852-t853-t854-t855-t856-t857-t858-t859-t860-t861-t862-t863-t864-t865-t866-t867-t868-t869-t870-t871-t872-t873-t874-t875-t876-t877-t878-t879-t880-t881-t882-t883-t884-t885-t886-t887-t888-t889-t890-t891-t892-t893-t894-t895-t896-t897-t898-t899-t900-t901-t902-t903-t904-t905-t906-t907-t908-t909-t910-t911-t912-t913-t914-t915-t916-t917-t918-t919-t920-t921-t922-t923-t924-t925-t926-t927-t928-t929-t930-t931-t932-t933-t934-t935-t936-t937-t938-t939-t940-t941-t942-t943-t944-t945-t946-t947-t948-t949-t950-t951-t952-t953-t954-t955-t956-t957-t958-t959-t960-t961-t962-t963-t964-t965-t966-t967-t968-t969-t970-t971-t972-t973-t974-t975-t976-t977-t978-t979-t980-t981-t982-t983-t984-t985-t986-t987-t988-t989-t990-t991-t992-t993-t994-t995-t996-t997-t998-t999-t1000-t1001-t1002-t1003-t1004-t1005-t1006-t1007-t1008-t1009-t1010-t1011-t1012-t1013-t1014-t1015-t1016-t1017-t1018-t1019-t1020-t1021-t1022-t1023-t1024-t1025-t1026-t1027-t1028-t1029-t1030-t1031-t1032-t1033-t1034-t1035-t1036-t1037-t1038-t1039-t1040-t1041-t1042-t1043-t1044-t1045-t1046-t1047-t1048-t1049-t1050-t1051-t1052-t1053-t1054-t1055-t1056-t1057-t1058-t1059-t1060-t1061-t1062-t1063-t1064-t1065-t1066-t1067-t1068-t1069-t1070-t1071-t1072-t1073-t1074-t1075-t1076-t1077-t1078-t1079-t1080-t1081-t1082-t1083-t1084-t1085-t1086-t1087-t1088-t1089-t1090-t1091-t1092-t1093-t1094-t1095-t1096-t1097-t1098-t1099-t1100-t1101-t1102-t1103-t1104-t1105-t1106-t1107-t1108-t1109-t1110-t1111-t1112-t1113-t1114-t1115-t1116-t1117-t1118-t1119-t1120-t1121-t1122-t1123-t1124-t1125-t1126-t1127-t1128-t1129-t1130-t1131-t1132-t1133-t1134-t1135-t1136-t1137-t1138-t1139-t1140-t1141-t1142-t1143-t1144-t1145-t1146-t1147-t1148-t1149-t1150-t1151-t1152-t1153-t1154-t1155-t1156-t1157-t1158-t1159-t1160-t1161-t1162-t1163-t1164-t1165-t1166-t1167-t1168-t1169-t1170-t1171-t1172-t1173-t1174-t1175-t1176-t1177-t1178-t1179-t1180-t1181-t1182-t1183-t1184-t1185-t1186-t1187-t1188-t1189-t1190-t1191-t1192-t1193-t1194-t1195-t1196-t1197-t1198-t1199-t1200-t1201-t1202-t1203-t1204-t1205-t1206-t1207-t1208-t1209-t1210-t1211;
t1212 = t252.*t630;
t631 = t36-t1212;
t632 = sqrt(real(abs(t631)));
t1213 = F_13.*t2;
t1214 = F_13.*t3;
t1215 = F_13.*t4;
t1216 = F_13.*t5;
t1217 = CMC1.*CMC3.*F1;
t1218 = CMC2.*CMC3.*F2;
t1219 = CMC1.*F1.*F3;
t1220 = CMC2.*F2.*F3;
t1221 = CMC1.*F3.*F_11;
t1222 = CMC3.*F1.*F_11;
t1223 = CMC2.*F3.*F_12;
t1224 = CMC3.*F2.*F_12;
t1275 = CMC3.*t4;
t1276 = CMC3.*t5;
t1277 = CMC1.*CMC3.*F_11;
t1278 = CMC2.*CMC3.*F_12;
t1279 = CMC1.*F1.*F_13.*2.0;
t1280 = CMC2.*F2.*F_13.*2.0;
t1281 = F1.*F3.*F_11;
t1282 = F2.*F3.*F_12;
t1225 = -t25-t26+t1213+t1214+t1215+t1216+t1217+t1218+t1219+t1220+t1221+t1222+t1223+t1224-t1275-t1276-t1277-t1278-t1279-t1280-t1281-t1282;
t1226 = 1.0./t1225;
t1227 = CMC1.*F3.*t6;
t1228 = F1.*F_13.*t4;
t1229 = CMC1.*CMC3.*t4;
t1230 = CMC1.*F3.*t4;
t1231 = CMC1.*F3.*t5;
t1232 = F1.*F3.*t7;
t1233 = CMC3.*F_11.*t4;
t1234 = F1.*F_13.*t2;
t1235 = F1.*F_13.*t3;
t1236 = CMC3.*F_11.*t6.*2.0;
t1237 = F1.*F_13.*t5;
t1238 = F1.*F_13.*t6;
t1239 = CMC3.*F1.*t8;
t1240 = CMC1.*F_13.*t8;
t1241 = F3.*F_11.*t8;
t1242 = CMC2.*CMC3.*F1.*F2;
t1243 = CMC1.*CMC2.*F3.*F_12;
t1244 = CMC1.*CMC3.*F3.*F_13;
t1245 = CMC1.*F1.*F3.*F_11;
t1246 = CMC2.*F2.*F3.*F_11.*2.0;
t1247 = CMC3.*F1.*F2.*F_12;
t1248 = t1227+t1228+t1229+t1230+t1231+t1232+t1233+t1234+t1235+t1236+t1237+t1238+t1239+t1240+t1241+t1242+t1243+t1244+t1245+t1246+t1247-CMC1.*CMC3.*t6-CMC3.*F1.*t4-CMC3.*F1.*t5-CMC3.*F1.*t6-CMC1.*F3.*t8-CMC1.*F_13.*t4.*2.0-CMC1.*F_13.*t6-CMC3.*F_11.*t8-F1.*F3.*t2-F3.*F_11.*t3-F3.*F_11.*t4-F3.*F_11.*t5-F3.*F_11.*t6-F3.*F_11.*t7-F1.*F_13.*t8-CMC1.*CMC2.*F2.*F3-CMC1.*CMC3.*F1.*F_11-CMC2.*CMC3.*F1.*F_12-CMC1.*F2.*F3.*F_12-CMC2.*F1.*F2.*F_13.*2.0-CMC3.*F1.*F3.*F_13;
t1249 = 1.0./t9;
t1250 = t2.*t632;
t1251 = t3.*t632;
t1252 = t7.*t632;
t1253 = t4.*t632;
t1254 = t5.*t632;
t1255 = t6.*t632;
t1257 = t25+t26-t27+t28+t29+t30+t31-t32-t33-t34+F3.*t6;
t1258 = t1257.^2;
t1259 = t24.*t1258;
t1260 = -t1212+t1259;
t1261 = sqrt(real(abs(t1260)));
t1262 = F_11.*t3;
t1263 = F_11.*t7;
t1264 = F_11.*t5;
t1265 = F_11.*t6;
t1266 = CMC1.*CMC2.*F2;
t1267 = CMC1.*CMC3.*F3;
t1268 = CMC2.*F1.*F2;
t1269 = CMC3.*F1.*F3;
t1270 = CMC1.*F2.*F_12;
t1271 = CMC2.*F1.*F_12;
t1272 = CMC1.*F3.*F_13;
t1273 = CMC3.*F1.*F_13;
t1274 = t1262+t1263+t1264+t1265+t1266+t1267+t1268+t1269+t1270+t1271+t1272+t1273-CMC1.*t5-CMC1.*t6-F1.*t3-F1.*t7-CMC1.*CMC2.*F_12-CMC1.*CMC3.*F_13-CMC2.*F2.*F_11.*2.0-CMC3.*F3.*F_11.*2.0-F1.*F2.*F_12-F1.*F3.*F_13;
t1283 = CMC1.*F1.*t1261.*2.0;
t1284 = CMC2.*F2.*t1261.*2.0;
t1285 = CMC3.*F3.*t1261.*2.0;
x_sol = [t1248./(t1213+t1214+t1215+t1216+t1217+t1218+t1219+t1220+t1221+t1222+t1223+t1224-CMC3.*t4-CMC3.*t5-F3.*t2-F3.*t3-CMC1.*CMC3.*F_11-CMC2.*CMC3.*F_12-CMC1.*F1.*F_13.*2.0-CMC2.*F2.*F_13.*2.0-F1.*F3.*F_11-F2.*F3.*F_12)+t1226.*t1249.*t1274.*(t25+t26-t27+t28+t29+t30+t31-t32-t33-t34+t1250+t1251+t1252+t1253+t1254+t1255+F3.*t6-CMC1.*F1.*t632.*2.0-CMC2.*F2.*t632.*2.0-CMC3.*F3.*t632.*2.0);t1226.*t1248+t1226.*t1249.*t1274.*(t25+t26-t27+t28+t29+t30+t31-t32-t33-t34-t1250-t1251-t1252-t1253-t1254-t1255+t1256+t1283+t1284+t1285)];
if nargout > 1
    t1286 = CMC2.*F3.*t6;
    t1287 = F2.*F_13.*t5;
    t1288 = CMC2.*CMC3.*t5;
    t1289 = CMC2.*F3.*t4;
    t1290 = CMC2.*F3.*t5;
    t1291 = F2.*F3.*t7;
    t1292 = F2.*F_13.*t2;
    t1293 = CMC3.*F_12.*t5;
    t1294 = F2.*F_13.*t3;
    t1295 = CMC3.*F_12.*t6.*2.0;
    t1296 = F2.*F_13.*t4;
    t1297 = F2.*F_13.*t6;
    t1298 = CMC3.*F2.*t8;
    t1299 = CMC2.*F_13.*t8;
    t1300 = F3.*F_12.*t8;
    t1301 = CMC1.*CMC3.*F1.*F2;
    t1302 = CMC1.*CMC2.*F3.*F_11;
    t1303 = CMC2.*CMC3.*F3.*F_13;
    t1304 = CMC1.*F1.*F3.*F_12.*2.0;
    t1305 = CMC3.*F1.*F2.*F_11;
    t1306 = CMC2.*F2.*F3.*F_12;
    t1307 = t1286+t1287+t1288+t1289+t1290+t1291+t1292+t1293+t1294+t1295+t1296+t1297+t1298+t1299+t1300+t1301+t1302+t1303+t1304+t1305+t1306-CMC2.*CMC3.*t6-CMC3.*F2.*t4-CMC3.*F2.*t5-CMC3.*F2.*t6-CMC2.*F3.*t8-CMC2.*F_13.*t5.*2.0-CMC2.*F_13.*t6-CMC3.*F_12.*t8-F2.*F3.*t3-F3.*F_12.*t2-F3.*F_12.*t4-F3.*F_12.*t5-F3.*F_12.*t6-F3.*F_12.*t7-F2.*F_13.*t8-CMC1.*CMC2.*F1.*F3-CMC1.*CMC3.*F2.*F_11-CMC2.*CMC3.*F2.*F_12-CMC1.*F1.*F2.*F_13.*2.0-CMC2.*F1.*F3.*F_11-CMC3.*F2.*F3.*F_13;
    t1308 = t1226.*t1307;
    t1309 = t2.*t1261;
    t1310 = t3.*t1261;
    t1311 = t7.*t1261;
    t1312 = t4.*t1261;
    t1313 = t5.*t1261;
    t1314 = t6.*t1261;
    t1315 = F_12.*t2;
    t1316 = F_12.*t7;
    t1317 = F_12.*t4;
    t1318 = F_12.*t6;
    t1319 = CMC1.*CMC2.*F1;
    t1320 = CMC2.*CMC3.*F3;
    t1321 = CMC1.*F1.*F2;
    t1322 = CMC3.*F2.*F3;
    t1323 = CMC1.*F2.*F_11;
    t1324 = CMC2.*F1.*F_11;
    t1325 = CMC2.*F3.*F_13;
    t1326 = CMC3.*F2.*F_13;
    t1327 = t1315+t1316+t1317+t1318+t1319+t1320+t1321+t1322+t1323+t1324+t1325+t1326-CMC2.*t4-CMC2.*t6-F2.*t2-F2.*t7-CMC1.*CMC2.*F_11-CMC2.*CMC3.*F_13-CMC1.*F1.*F_12.*2.0-CMC3.*F3.*F_12.*2.0-F1.*F2.*F_11-F2.*F3.*F_13;
    t1328 = t25+t26-t27+t28+t29+t30+t31-t32-t33-t34-t1283-t1284-t1285+t1309+t1310+t1311+t1312+t1313+t1314+F3.*t6;
    y_sol = [t1308+t1226.*t1249.*t1327.*t1328;t1308+t1226.*t1249.*t1327.*(t25+t26-t27+t28+t29+t30+t31-t32-t33-t34+t1256+t1283+t1284+t1285-t1309-t1310-t1311-t1312-t1313-t1314)];
end
if nargout > 2
    z_sol = [t1249.*t1328;t1249.*(t25+t26-t27+t28+t29+t30+t31-t32-t33-t34+t1256+t1283+t1284+t1285-t1309-t1310-t1311-t1312-t1313-t1314)];
end
